simulink model "Quadcopter_v5_1_full"  (R2021a)
settings: Solver=ode4  StartTime=0.0  StopTime=87  FixedStep=0.001  RelTol=1e-6
values from neighbouring files (symbols this model uses):
  mean_wind = [2.72 , 1.75, -0.006]    [main_run.m]    (also in main_run_5_1.m; param_est.m = [2.72 , 1.75, .006])
  q = X(7:10)    [EKF_without_wind.m]
  r = linspace(floor(nr*0.01)/nr,1,nr)    [main_run.m]    (also in main_run_5_1.m)
  w1 = w(1)    [EKF_without_wind.m]
  x0 = [0,0,0,1,0,0,0,-P.mean_wind,0,0,0]    [main_run.m]    (also in main_run_5_1.m)
  xref = [1,1,-8,1,0,0,0,-P.mean_wind]    [main_run.m]    (also in main_run_5_1.m)
undefined symbols (not defined in the file or in its folder): HDBK, MIL, Moderate, P, u1, v1
libraries: simulink x1, aerolibwind2 x1
(part 3 of 6)

== matlab function Quadcopter_v5_1_full/Controller /State Dependent LQR/LQR ==
  data: x input; r input; y output; P parameter; u_c input; t input
function y  = LQR_state(x, r,P,u_c, t)
%State dependent LQR 

  %inputs
  %x---states; this will give all states, f_c and omega
  %prev_state---states from last time step
  %sumError-- not need
  %ref--- reference
y=zeros(4,1);


K0=zeros(4,10);
coder.extrinsic('lqr')

xref= r(1:10);
x_c=x(1:10);
uref = P.uref;


D = P.D;
m = P.m;

p = reshape(x_c(1:3),[3 1]);
q = reshape(x_c(4:7),[4 1]);
v = reshape(x_c(8:10),[3 1]);
nq = norm(q);
% q*q.'
ddqu_dq = (eye(4) - (nq^-2)*q*q.')*(nq^-1) ;

if t==0
    c = uref(4);
    wx = uref(1);
    wy = uref(2);
    wz = uref(3);
else
    c = u_c(4);
    wx = u_c(1);
    wy = u_c(2);
    wz = u_c(3);

end 


qw = q(1);
qx = q(2);
qy = q(3);
qz = q(4);

ddp_dv = eye([3 3]);
ddq_dq = 0.5*[ 0, -wx, -wy, -wz;...
              wx,   0,  wz, -wy;...
              wy, -wz,   0,  wx;...
              wz,  wy, -wx,   0]*ddqu_dq;
ddq_dw = 0.5*[-qx, -qy, -qz;...
               qw, -qz, -qy;...
               qz,  qw,  qx;...
              -qy,  qx,  qw];
ddc_dq = 2*c*[ qy,  qz,  qw, qx;...
              -qx, -qw,  qz, qy;...
               qw, -qx, -qy, qz]*ddqu_dq;
ddv_dc = -[            qw*qy + qx*qz;...
                      qy*qz - qw*qx;...
          qw^2 - qx^2 - qy^2 + qz^2]; 
      
R=quater_rot(q);

% ddrg_v= -(R*D*R'*(norm(v)*eye(3)+(v*v')/norm(v)))/m; %also jacobian of vdot wrt v     
% vx=v(1);
% vy=v(2);
% vz=v(3);
% dx=D(1);
% dy=D(2);
% dz=D(3);
% ddrg_q=[ ((qw^2/(abs(qw)^2 + abs(qx)^2 + abs(qy)^2 + abs(qz)^2) - 1)*(vy*(2*dy*qw*(2*qw*qz - 2*qx*qy)*(abs(vx)^2 + abs(vy)^2 + abs(vz)^2)^(1/2) - 2*dx*qw*(2*qw*qz + 2*qx*qy)*(abs(vx)^2 + abs(vy)^2 + abs(vz)^2)^(1/2) + 2*dz*qx*(2*qw*qy + 2*qx*qz)*(abs(vx)^2 + abs(vy)^2 + abs(vz)^2)^(1/2) + 2*dz*qy*(2*qw*qx - 2*qy*qz)*(abs(vx)^2 + abs(vy)^2 + abs(vz)^2)^(1/2) - 2*dx*qz*(abs(vx)^2 + abs(vy)^2 + abs(vz)^2)^(1/2)*(qw^2 + qx^2 - qy^2 - qz^2) + 2*dy*qz*(abs(vx)^2 + abs(vy)^2 + abs(vz)^2)^(1/2)*(qw^2 - qx^2 + qy^2 - qz^2)) + vz*(2*dx*qw*(2*qw*qy - 2*qx*qz)*(abs(vx)^2 + abs(vy)^2 + abs(vz)^2)^(1/2) + 2*dy*qx*(2*qw*qz - 2*qx*qy)*(abs(vx)^2 + abs(vy)^2 + abs(vz)^2)^(1/2) - 2*dz*qw*(2*qw*qy + 2*qx*qz)*(abs(vx)^2 + abs(vy)^2 + abs(vz)^2)^(1/2) + 2*dy*qz*(2*qw*qx + 2*qy*qz)*(abs(vx)^2 + abs(vy)^2 + abs(vz)^2)^(1/2) + 2*dx*qy*(abs(vx)^2 + abs(vy)^2 + abs(vz)^2)^(1/2)*(qw^2 + qx^2 - qy^2 - qz^2) - 2*dz*qy*(abs(vx)^2 + abs(vy)^2 + abs(vz)^2)^(1/2)*(qw^2 - qx^2 - qy^2 + qz^2)) - vx*(4*dy*qz*(2*qw*qz - 2*qx*qy)*(abs(vx)^2 + abs(vy)^2 + abs(vz)^2)^(1/2) + 4*dz*qy*(2*qw*qy + 2*qx*qz)*(abs(vx)^2 + abs(vy)^2 + abs(vz)^2)^(1/2) + 4*dx*qw*(abs(vx)^2 + abs(vy)^2 + abs(vz)^2)^(1/2)*(qw^2 + qx^2 - qy^2 - qz^2))))/(abs(qw)^2 + abs(qx)^2 + abs(qy)^2 + abs(qz)^2)^(1/2) + (qw*qy*(vy*(2*dx*qy*(2*qw*qz + 2*qx*qy)*(abs(vx)^2 + abs(vy)^2 + abs(vz)^2)^(1/2) + 2*dz*qw*(2*qw*qx - 2*qy*qz)*(abs(vx)^2 + abs(vy)^2 + abs(vz)^2)^(1/2) + 2*dy*qy*(2*qw*qz - 2*qx*qy)*(abs(vx)^2 + abs(vy)^2 + abs(vz)^2)^(1/2) - 2*dz*qz*(2*qw*qy + 2*qx*qz)*(abs(vx)^2 + abs(vy)^2 + abs(vz)^2)^(1/2) - 2*dx*qx*(abs(vx)^2 + abs(vy)^2 + abs(vz)^2)^(1/2)*(qw^2 + qx^2 - qy^2 - qz^2) - 2*dy*qx*(abs(vx)^2 + abs(vy)^2 + abs(vz)^2)^(1/2)*(qw^2 - qx^2 + qy^2 - qz^2)) - vz*(2*dx*qy*(2*qw*qy - 2*qx*qz)*(abs(vx)^2 + abs(vy)^2 + abs(vz)^2)^(1/2) + 2*dy*qx*(2*qw*qx + 2*qy*qz)*(abs(vx)^2 + abs(vy)^2 + abs(vz)^2)^(1/2) - 2*dy*qz*(2*qw*qz - 2*qx*qy)*(abs(vx)^2 + abs(vy)^2 + abs(vz)^2)^(1/2) - 2*dz*qy*(2*qw*qy + 2*qx*qz)*(abs(vx)^2 + abs(vy)^2 + abs(vz)^2)^(1/2) - 2*dx*qw*(abs(vx)^2 + abs(vy)^2 + abs(vz)^2)^(1/2)*(qw^2 + qx^2 - qy^2 - qz^2) + 2*dz*qw*(abs(vx)^2 + abs(vy)^2 + abs(vz)^2)^(1/2)*(qw^2 - qx^2 - qy^2 + qz^2)) + vx*(4*dy*qx*(2*qw*qz - 2*qx*qy)*(abs(vx)^2 + abs(vy)^2 + abs(vz)^2)^(1/2) - 4*dz*qw*(2*qw*qy + 2*qx*qz)*(abs(vx)^2 + abs(vy)^2 + abs(vz)^2)^(1/2) + 4*dx*qy*(abs(vx)^2 + abs(vy)^2 + abs(vz)^2)^(1/2)*(qw^2 + qx^2 - qy^2 - qz^2))))/(abs(qw)^2 + abs(qx)^2 + abs(qy)^2 + abs(qz)^2)^(3/2) - (qw*qx*(vy*(2*dx*qx*(2*qw*qz + 2*qx*qy)*(abs(vx)^2 + abs(vy)^2 + abs(vz)^2)^(1/2) + 2*dy*qx*(2*qw*qz - 2*qx*qy)*(abs(vx)^2 + abs(vy)^2 + abs(vz)^2)^(1/2) - 2*dz*qw*(2*qw*qy + 2*qx*qz)*(abs(vx)^2 + abs(vy)^2 + abs(vz)^2)^(1/2) - 2*dz*qz*(2*qw*qx - 2*qy*qz)*(abs(vx)^2 + abs(vy)^2 + abs(vz)^2)^(1/2) + 2*dx*qy*(abs(vx)^2 + abs(vy)^2 + abs(vz)^2)^(1/2)*(qw^2 + qx^2 - qy^2 - qz^2) + 2*dy*qy*(abs(vx)^2 + abs(vy)^2 + abs(vz)^2)^(1/2)*(qw^2 - qx^2 + qy^2 - qz^2)) - vz*(2*dx*qx*(2*qw*qy - 2*qx*qz)*(abs(vx)^2 + abs(vy)^2 + abs(vz)^2)^(1/2) + 2*dy*qw*(2*qw*qz - 2*qx*qy)*(abs(vx)^2 + abs(vy)^2 + abs(vz)^2)^(1/2) - 2*dy*qy*(2*qw*qx + 2*qy*qz)*(abs(vx)^2 + abs(vy)^2 + abs(vz)^2)^(1/2) + 2*dz*qx*(2*qw*qy + 2*qx*qz)*(abs(vx)^2 + abs(vy)^2 + abs(vz)^2)^(1/2) - 2*dx*qz*(abs(vx)^2 + abs(vy)^2 + abs(vz)^2)^(1/2)*(qw^2 + qx^2 - qy^2 - qz^2) - 2*dz*qz*(abs(vx)^2 + abs(vy)^2 + abs(vz)^2)^(1/2)*(qw^2 - qx^2 - qy^2 + qz^2)) + vx*(4*dz*qz*(2*qw*qy + 2*qx*qz)*(abs(vx)^2 + abs(vy)^2 + abs(vz)^2)^(1/2) - 4*dy*qy*(2*qw*qz - 2*qx*qy)*(abs(vx)^2 + abs(vy)^2 + abs(vz)^2)^(1/2) + 4*dx*qx*(abs(vx)^2 + abs(vy)^2 + abs(vz)^2)^(1/2)*(qw^2 + qx^2 - qy^2 - qz^2))))/(abs(qw)^2 + abs(qx)^2 + abs(qy)^2 + abs(qz)^2)^(3/2) - (qw*qz*(vz*(2*dx*qz*(2*qw*qy - 2*qx*qz)*(abs(vx)^2 + abs(vy)^2 + abs(vz)^2)^(1/2) - 2*dy*qw*(2*qw*qx + 2*qy*qz)*(abs(vx)^2 + abs(vy)^2 + abs(vz)^2)^(1/2) - 2*dy*qy*(2*qw*qz - 2*qx*qy)*(abs(vx)^2 + abs(vy)^2 + abs(vz)^2)^(1/2) + 2*dz*qz*(2*qw*qy + 2*qx*qz)*(abs(vx)^2 + abs(vy)^2 + abs(vz)^2)^(1/2) + 2*dx*qx*(abs(vx)^2 + abs(vy)^2 + abs(vz)^2)^(1/2)*(qw^2 + qx^2 - qy^2 - qz^2) + 2*dz*qx*(abs(vx)^2 + abs(vy)^2 + abs(vz)^2)^(1/2)*(qw^2 - qx^2 - qy^2 + qz^2)) - vy*(2*dx*qz*(2*qw*qz + 2*qx*qy)*(abs(vx)^2 + abs(vy)^2 + abs(vz)^2)^(1/2) + 2*dz*qx*(2*qw*qx - 2*qy*qz)*(abs(vx)^2 + abs(vy)^2 + abs(vz)^2)^(1/2) - 2*dy*qz*(2*qw*qz - 2*qx*qy)*(abs(vx)^2 + abs(vy)^2 + abs(vz)^2)^(1/2) - 2*dz*qy*(2*qw*qy + 2*qx*qz)*(abs(vx)^2 + abs(vy)^2 + abs(vz)^2)^(1/2) - 2*dx*qw*(abs(vx)^2 + abs(vy)^2 + abs(vz)^2)^(1/2)*(qw^2 + qx^2 - qy^2 - qz^2) + 2*dy*qw*(abs(vx)^2 + abs(vy)^2 + abs(vz)^2)^(1/2)*(qw^2 - qx^2 + qy^2 - qz^2)) + vx*(4*dy*qw*(2*qw*qz - 2*qx*qy)*(abs(vx)^2 + abs(vy)^2 + abs(vz)^2)^(1/2) + 4*dz*qx*(2*qw*qy + 2*qx*qz)*(abs(vx)^2 + abs(vy)^2 + abs(vz)^2)^(1/2) - 4*dx*qz*(abs(vx)^2 + abs(vy)^2 + abs(vz)^2)^(1/2)*(qw^2 + qx^2 - qy^2 - qz^2))))/(abs(qw)^2 + abs(qx)^2 + abs(qy)^2 + abs(qz)^2)^(3/2), (qw*qx*(vy*(2*dy*qw*(2*qw*qz - 2*qx*qy)*(abs(vx)^2 + abs(vy)^2 + abs(vz)^2)^(1/2) - 2*dx*qw*(2*qw*qz + 2*qx*qy)*(abs(vx)^2 + abs(vy)^2 + abs(vz)^2)^(1/2) + 2*dz*qx*(2*qw*qy + 2*qx*qz)*(abs(vx)^2 + abs(vy)^2 + abs(vz)^2)^(1/2) + 2*dz*qy*(2*qw*qx - 2*qy*qz)*(abs(vx)^2 + abs(vy)^2 + abs(vz)^2)^(1/2) - 2*dx*qz*(abs(vx)^2 + abs(vy)^2 + abs(vz)^2)^(1/2)*(qw^2 + qx^2 - qy^2 - qz^2) + 2*dy*qz*(abs(vx)^2 + abs(vy)^2 + abs(vz)^2)^(1/2)*(qw^2 - qx^2 + qy^2 - qz^2)) + vz*(2*dx*qw*(2*qw*qy - 2*qx*qz)*(abs(vx)^2 + abs(vy)^2 + abs(vz)^2)^(1/2) + 2*dy*qx*(2*qw*qz - 2*qx*qy)*(abs(vx)^2 + abs(vy)^2 + abs(vz)^2)^(1/2) - 2*dz*qw*(2*qw*qy + 2*qx*qz)*(abs(vx)^2 + abs(vy)^2 + abs(vz)^2)^(1/2) + 2*dy*qz*(2*qw*qx + 2*qy*qz)*(abs(vx)^2 + abs(vy)^2 + abs(vz)^2)^(1/2) + 2*dx*qy*(abs(vx)^2 + abs(vy)^2 + abs(vz)^2)^(1/2)*(qw^2 + qx^2 - qy^2 - qz^2) - 2*dz*qy*(abs(vx)^2 + abs(vy)^2 + abs(vz)^2)^(1/2)*(qw^2 - qx^2 - qy^2 + qz^2)) - vx*(4*dy*qz*(2*qw*qz - 2*qx*qy)*(abs(vx)^2 + abs(vy)^2 + abs(vz)^2)^(1/2) + 4*dz*qy*(2*qw*qy + 2*qx*qz)*(abs(vx)^2 + abs(vy)^2 + abs(vz)^2)^(1/2) + 4*dx*qw*(abs(vx)^2 + abs(vy)^2 + abs(vz)^2)^(1/2)*(qw^2 + qx^2 - qy^2 - qz^2))))/(abs(qw)^2 + abs(qx)^2 + abs(qy)^2 + abs(qz)^2)^(3/2) - ((qx^2/(abs(qw)^2 + abs(qx)^2 + abs(qy)^2 + abs(qz)^2) - 1)*(vy*(2*dx*qx*(2*qw*qz + 2*qx*qy)*(abs(vx)^2 + abs(vy)^2 + abs(vz)^2)^(1/2) + 2*dy*qx*(2*qw*qz - 2*qx*qy)*(abs(vx)^2 + abs(vy)^2 + abs(vz)^2)^(1/2) - 2*dz*qw*(2*qw*qy + 2*qx*qz)*(abs(vx)^2 + abs(vy)^2 + abs(vz)^2)^(1/2) - 2*dz*qz*(2*qw*qx - 2*qy*qz)*(abs(vx)^2 + abs(vy)^2 + abs(vz)^2)^(1/2) + 2*dx*qy*(abs(vx)^2 + abs(vy)^2 + abs(vz)^2)^(1/2)*(qw^2 + qx^2 - qy^2 - qz^2) + 2*dy*qy*(abs(vx)^2 + abs(vy)^2 + abs(vz)^2)^(1/2)*(qw^2 - qx^2 + qy^2 - qz^2)) - vz*(2*dx*qx*(2*qw*qy - 2*qx*qz)*(abs(vx)^2 + abs(vy)^2 + abs(vz)^2)^(1/2) + 2*dy*qw*(2*qw*qz - 2*qx*qy)*(abs(vx)^2 + abs(vy)^2 + abs(vz)^2)^(1/2) - 2*dy*qy*(2*qw*qx + 2*qy*qz)*(abs(vx)^2 + abs(vy)^2 + abs(vz)^2)^(1/2) + 2*dz*qx*(2*qw*qy + 2*qx*qz)*(abs(vx)^2 + abs(vy)^2 + abs(vz)^2)^(1/2) - 2*dx*qz*(abs(vx)^2 + abs(vy)^2 + abs(vz)^2)^(1/2)*(qw^2 + qx^2 - qy^2 - qz^2) - 2*dz*qz*(abs(vx)^2 + abs(vy)^2 + abs(vz)^2)^(1/2)*(qw^2 - qx^2 - qy^2 + qz^2)) + vx*(4*dz*qz*(2*qw*qy + 2*qx*qz)*(abs(vx)^2 + abs(vy)^2 + abs(vz)^2)^(1/2) - 4*dy*qy*(2*qw*qz - 2*qx*qy)*(abs(vx)^2 + abs(vy)^2 + abs(vz)^2)^(1/2) + 4*dx*qx*(abs(vx)^2 + abs(vy)^2 + abs(vz)^2)^(1/2)*(qw^2 + qx^2 - qy^2 - qz^2))))/(abs(qw)^2 + abs(qx)^2 + abs(qy)^2 + abs(qz)^2)^(1/2) + (qx*qy*(vy*(2*dx*qy*(2*qw*qz + 2*qx*qy)*(abs(vx)^2 + abs(vy)^2 + abs(vz)^2)^(1/2) + 2*dz*qw*(2*qw*qx - 2*qy*qz)*(abs(vx)^2 + abs(vy)^2 + abs(vz)^2)^(1/2) + 2*dy*qy*(2*qw*qz - 2*qx*qy)*(abs(vx)^2 + abs(vy)^2 + abs(vz)^2)^(1/2) - 2*dz*qz*(2*qw*qy + 2*qx*qz)*(abs(vx)^2 + abs(vy)^2 + abs(vz)^2)^(1/2) - 2*dx*qx*(abs(vx)^2 + abs(vy)^2 + abs(vz)^2)^(1/2)*(qw^2 + qx^2 - qy^2 - qz^2) - 2*dy*qx*(abs(vx)^2 + abs(vy)^2 + abs(vz)^2)^(1/2)*(qw^2 - qx^2 + qy^2 - qz^2)) - vz*(2*dx*qy*(2*qw*qy - 2*qx*qz)*(abs(vx)^2 + abs(vy)^2 + abs(vz)^2)^(1/2) + 2*dy*qx*(2*qw*qx + 2*qy*qz)*(abs(vx)^2 + abs(vy)^2 + abs(vz)^2)^(1/2) - 2*dy*qz*(2*qw*qz - 2*qx*qy)*(abs(vx)^2 + abs(vy)^2 + abs(vz)^2)^(1/2) - 2*dz*qy*(2*qw*qy + 2*qx*qz)*(abs(vx)^2 + abs(vy)^2 + abs(vz)^2)^(1/2) - 2*dx*qw*(abs(vx)^2 + abs(vy)^2 + abs(vz)^2)^(1/2)*(qw^2 + qx^2 - qy^2 - qz^2) + 2*dz*qw*(abs(vx)^2 + abs(vy)^2 + abs(vz)^2)^(1/2)*(qw^2 - qx^2 - qy^2 + qz^2)) + vx*(4*dy*qx*(2*qw*qz - 2*qx*qy)*(abs(vx)^2 + abs(vy)^2 + abs(vz)^2)^(1/2) - 4*dz*qw*(2*qw*qy + 2*qx*qz)*(abs(vx)^2 + abs(vy)^2 + abs(vz)^2)^(1/2) + 4*dx*qy*(abs(vx)^2 + abs(vy)^2 + abs(vz)^2)^(1/2)*(qw^2 + qx^2 - qy^2 - qz^2))))/(abs(qw)^2 + abs(qx)^2 + abs(qy)^2 + abs(qz)^2)^(3/2) - (qx*qz*(vz*(2*dx*qz*(2*qw*qy - 2*qx*qz)*(abs(vx)^2 + abs(vy)^2 + abs(vz)^2)^(1/2) - 2*dy*qw*(2*qw*qx + 2*qy*qz)*(abs(vx)^2 + abs(vy)^2 + abs(vz)^2)^(1/2) - 2*dy*qy*(2*qw*qz - 2*qx*qy)*(abs(vx)^2 + abs(vy)^2 + abs(vz)^2)^(1/2) + 2*dz*qz*(2*qw*qy + 2*qx*qz)*(abs(vx)^2 + abs(vy)^2 + abs(vz)^2)^(1/2) + 2*dx*qx*(abs(vx)^2 + abs(vy)^2 + abs(vz)^2)^(1/2)*(qw^2 + qx^2 - qy^2 - qz^2) + 2*dz*qx*(abs(vx)^2 + abs(vy)^2 + abs(vz)^2)^(1/2)*(qw^2 - qx^2 - qy^2 + qz^2)) - vy*(2*dx*qz*(2*qw*qz + 2*qx*qy)*(abs(vx)^2 + abs(vy)^2 + abs(vz)^2)^(1/2) + 2*dz*qx*(2*qw*qx - 2*qy*qz)*(abs(vx)^2 + abs(vy)^2 + abs(vz)^2)^(1/2) - 2*dy*qz*(2*qw*qz - 2*qx*qy)*(abs(vx)^2 + abs(vy)^2 + abs(vz)^2)^(1/2) - 2*dz*qy*(2*qw*qy + 2*qx*qz)*(abs(vx)^2 + abs(vy)^2 + abs(vz)^2)^(1/2) - 2*dx*qw*(abs(vx)^2 + abs(vy)^2 + abs(vz)^2)^(1/2)*(qw^2 + qx^2 - qy^2 - qz^2) + 2*dy*qw*(abs(vx)^2 + abs(vy)^2 + abs(vz)^2)^(1/2)*(qw^2 - qx^2 + qy^2 - qz^2)) + vx*(4*dy*qw*(2*qw*qz - 2*qx*qy)*(abs(vx)^2 + abs(vy)^2 + abs(vz)^2)^(1/2) + 4*dz*qx*(2*qw*qy + 2*qx*qz)*(abs(vx)^2 + abs(vy)^2 + abs(vz)^2)^(1/2) - 4*dx*qz*(abs(vx)^2 + abs(vy)^2 + abs(vz)^2)^(1/2)*(qw^2 + qx^2 - qy^2 - qz^2))))/(abs(qw)^2 + abs(qx)^2 + abs(qy)^2 + abs(qz)^2)^(3/2), ((qy^2/(abs(qw)^2 + abs(qx)^2 + abs(qy)^2 + abs(qz)^2) - 1)*(vy*(2*dx*qy*(2*qw*qz + 2*qx*qy)*(abs(vx)^2 + abs(vy)^2 + abs(vz)^2)^(1/2) + 2*dz*qw*(2*qw*qx - 2*qy*qz)*(abs(vx)^2 + abs(vy)^2 + abs(vz)^2)^(1/2) + 2*dy*qy*(2*qw*qz - 2*qx*qy)*(abs(vx)^2 + abs(vy)^2 + abs(vz)^2)^(1/2) - 2*dz*qz*(2*qw*qy + 2*qx*qz)*(abs(vx)^2 + abs(vy)^2 + abs(vz)^2)^(1/2) - 2*dx*qx*(abs(vx)^2 + abs(vy)^2 + abs(vz)^2)^(1/2)*(qw^2 + qx^2 - qy^2 - qz^2) - 2*dy*qx*(abs(vx)^2 + abs(vy)^2 + abs(vz)^2)^(1/2)*(qw^2 - qx^2 + qy^2 - qz^2)) - vz*(2*dx*qy*(2*qw*qy - 2*qx*qz)*(abs(vx)^2 + abs(vy)^2 + abs(vz)^2)^(1/2) + 2*dy*qx*(2*qw*qx + 2*qy*qz)*(abs(vx)^2 + abs(vy)^2 + abs(vz)^2)^(1/2) - 2*dy*qz*(2*qw*qz - 2*qx*qy)*(abs(vx)^2 + abs(vy)^2 + abs(vz)^2)^(1/2) - 2*dz*qy*(2*qw*qy + 2*qx*qz)*(abs(vx)^2 + abs(vy)^2 + abs(vz)^2)^(1/2) - 2*dx*qw*(abs(vx)^2 + abs(vy)^2 + abs(vz)^2)^(1/2)*(qw^2 + qx^2 - qy^2 - qz^2) + 2*dz*qw*(abs(vx)^2 + abs(vy)^2 + abs(vz)^2)^(1/2)*(qw^2 - qx^2 - qy^2 + qz^2)) + vx*(4*dy*qx*(2*qw*qz - 2*qx*qy)*(abs(vx)^2 + abs(vy)^2 + abs(vz)^2)^(1/2) - 4*dz*qw*(2*qw*qy + 2*qx*qz)*(abs(vx)^2 + abs(vy)^2 + abs(vz)^2)^(1/2) + 4*dx*qy*(abs(vx)^2 + abs(vy)^2 + abs(vz)^2)^(1/2)*(qw^2 + qx^2 - qy^2 - qz^2))))/(abs(qw)^2 + abs(qx)^2 + abs(qy)^2 + abs(qz)^2)^(1/2) + (qw*qy*(vy*(2*dy*qw*(2*qw*qz - 2*qx*qy)*(abs(vx)^2 + abs(vy)^2 + abs(vz)^2)^(1/2) - 2*dx*qw*(2*qw*qz + 2*qx*qy)*(abs(vx)^2 + abs(vy)^2 + abs(vz)^2)^(1/2) + 2*dz*qx*(2*qw*qy + 2*qx*qz)*(abs(vx)^2 + abs(vy)^2 + abs(vz)^2)^(1/2) + 2*dz*qy*(2*qw*qx - 2*qy*qz)*(abs(vx)^2 + abs(vy)^2 + abs(vz)^2)^(1/2) - 2*dx*qz*(abs(vx)^2 + abs(vy)^2 + abs(vz)^2)^(1/2)*(qw^2 + qx^2 - qy^2 - qz^2) + 2*dy*qz*(abs(vx)^2 + abs(vy)^2 + abs(vz)^2)^(1/2)*(qw^2 - qx^2 + qy^2 - qz^2)) + vz*(2*dx*qw*(2*qw*qy - 2*qx*qz)*(abs(vx)^2 + abs(vy)^2 + abs(vz)^2)^(1/2) + 2*dy*qx*(2*qw*qz - 2*qx*qy)*(abs(vx)^2 + abs(vy)^2 + abs(vz)^2)^(1/2) - 2*dz*qw*(2*qw*qy + 2*qx*qz)*(abs(vx)^2 + abs(vy)^2 + abs(vz)^2)^(1/2) + 2*dy*qz*(2*qw*qx + 2*qy*qz)*(abs(vx)^2 + abs(vy)^2 + abs(vz)^2)^(1/2) + 2*dx*qy*(abs(vx)^2 + abs(vy)^2 + abs(vz)^2)^(1/2)*(qw^2 + qx^2 - qy^2 - qz^2) - 2*dz*qy*(abs(vx)^2 + abs(vy)^2 + abs(vz)^2)^(1/2)*(qw^2 - qx^2 - qy^2 + qz^2)) - vx*(4*dy*qz*(2*qw*qz - 2*qx*qy)*(abs(vx)^2 + abs(vy)^2 + abs(vz)^2)^(1/2) + 4*dz*qy*(2*qw*qy + 2*qx*qz)*(abs(vx)^2 + abs(vy)^2 + abs(vz)^2)^(1/2) + 4*dx*qw*(abs(vx)^2 + abs(vy)^2 + abs(vz)^2)^(1/2)*(qw^2 + qx^2 - qy^2 - qz^2))))/(abs(qw)^2 + abs(qx)^2 + abs(qy)^2 + abs(qz)^2)^(3/2) - (qx*qy*(vy*(2*dx*qx*(2*qw*qz + 2*qx*qy)*(abs(vx)^2 + abs(vy)^2 + abs(vz)^2)^(1/2) + 2*dy*qx*(2*qw*qz - 2*qx*qy)*(abs(vx)^2 + abs(vy)^2 + abs(vz)^2)^(1/2) - 2*dz*qw*(2*qw*qy + 2*qx*qz)*(abs(vx)^2 + abs(vy)^2 + abs(vz)^2)^(1/2) - 2*dz*qz*(2*qw*qx - 2*qy*qz)*(abs(vx)^2 + abs(vy)^2 + abs(vz)^2)^(1/2) + 2*dx*qy*(abs(vx)^2 + abs(vy)^2 + abs(vz)^2)^(1/2)*(qw^2 + qx^2 - qy^2 - qz^2) + 2*dy*qy*(abs(vx)^2 + abs(vy)^2 + abs(vz)^2)^(1/2)*(qw^2 - qx^2 + qy^2 - qz^2)) - vz*(2*dx*qx*(2*qw*qy - 2*qx*qz)*(abs(vx)^2 + abs(vy)^2 + abs(vz)^2)^(1/2) + 2*dy*qw*(2*qw*qz - 2*qx*qy)*(abs(vx)^2 + abs(vy)^2 + abs(vz)^2)^(1/2) - 2*dy*qy*(2*qw*qx + 2*qy*qz)*(abs(vx)^2 + abs(vy)^2 + abs(vz)^2)^(1/2) + 2*dz*qx*(2*qw*qy + 2*qx*qz)*(abs(vx)^2 + abs(vy)^2 + abs(vz)^2)^(1/2) - 2*dx*qz*(abs(vx)^2 + abs(vy)^2 + abs(vz)^2)^(1/2)*(qw^2 + qx^2 - qy^2 - qz^2) - 2*dz*qz*(abs(vx)^2 + abs(vy)^2 + abs(vz)^2)^(1/2)*(qw^2 - qx^2 - qy^2 + qz^2)) + vx*(4*dz*qz*(2*qw*qy + 2*qx*qz)*(abs(vx)^2 + abs(vy)^2 + abs(vz)^2)^(1/2) - 4*dy*qy*(2*qw*qz - 2*qx*qy)*(abs(vx)^2 + abs(vy)^2 + abs(vz)^2)^(1/2) + 4*dx*qx*(abs(vx)^2 + abs(vy)^2 + abs(vz)^2)^(1/2)*(qw^2 + qx^2 - qy^2 - qz^2))))/(abs(qw)^2 + abs(qx)^2 + abs(qy)^2 + abs(qz)^2)^(3/2) - (qy*qz*(vz*(2*dx*qz*(2*qw*qy - 2*qx*qz)*(abs(vx)^2 + abs(vy)^2 + abs(vz)^2)^(1/2) - 2*dy*qw*(2*qw*qx + 2*qy*qz)*(abs(vx)^2 + abs(vy)^2 + abs(vz)^2)^(1/2) - 2*dy*qy*(2*qw*qz - 2*qx*qy)*(abs(vx)^2 + abs(vy)^2 + abs(vz)^2)^(1/2) + 2*dz*qz*(2*qw*qy + 2*qx*qz)*(abs(vx)^2 + abs(vy)^2 + abs(vz)^2)^(1/2) + 2*dx*qx*(abs(vx)^2 + abs(vy)^2 + abs(vz)^2)^(1/2)*(qw^2 + qx^2 - qy^2 - qz^2) + 2*dz*qx*(abs(vx)^2 + abs(vy)^2 + abs(vz)^2)^(1/2)*(qw^2 - qx^2 - qy^2 + qz^2)) - vy*(2*dx*qz*(2*qw*qz + 2*qx*qy)*(abs(vx)^2 + abs(vy)^2 + abs(vz)^2)^(1/2) + 2*dz*qx*(2*qw*qx - 2*qy*qz)*(abs(vx)^2 + abs(vy)^2 + abs(vz)^2)^(1/2) - 2*dy*qz*(2*qw*qz - 2*qx*qy)*(abs(vx)^2 + abs(vy)^2 + abs(vz)^2)^(1/2) - 2*dz*qy*(2*qw*qy + 2*qx*qz)*(abs(vx)^2 + abs(vy)^2 + abs(vz)^2)^(1/2) - 2*dx*qw*(abs(vx)^2 + abs(vy)^2 + abs(vz)^2)^(1/2)*(qw^2 + qx^2 - qy^2 - qz^2) + 2*dy*qw*(abs(vx)^2 + abs(vy)^2 + abs(vz)^2)^(1/2)*(qw^2 - qx^2 + qy^2 - qz^2)) + vx*(4*dy*qw*(2*qw*qz - 2*qx*qy)*(abs(vx)^2 + abs(vy)^2 + abs(vz)^2)^(1/2) + 4*dz*qx*(2*qw*qy + 2*qx*qz)*(abs(vx)^2 + abs(vy)^2 + abs(vz)^2)^(1/2) - 4*dx*qz*(abs(vx)^2 + abs(vy)^2 + abs(vz)^2)^(1/2)*(qw^2 + qx^2 - qy^2 - qz^2))))/(abs(qw)^2 + abs(qx)^2 + abs(qy)^2 + abs(qz)^2)^(3/2), (qw*qz*(vy*(2*dy*qw*(2*qw*qz - 2*qx*qy)*(abs(vx)^2 + abs(vy)^2 + abs(vz)^2)^(1/2) - 2*dx*qw*(2*qw*qz + 2*qx*qy)*(abs(vx)^2 + abs(vy)^2 + abs(vz)^2)^(1/2) + 2*dz*qx*(2*qw*qy + 2*qx*qz)*(abs(vx)^2 + abs(vy)^2 + abs(vz)^2)^(1/2) + 2*dz*qy*(2*qw*qx - 2*qy*qz)*(abs(vx)^2 + abs(vy)^2 + abs(vz)^2)^(1/2) - 2*dx*qz*(abs(vx)^2 + abs(vy)^2 + abs(vz)^2)^(1/2)*(qw^2 + qx^2 - qy^2 - qz^2) + 2*dy*qz*(abs(vx)^2 + abs(vy)^2 + abs(vz)^2)^(1/2)*(qw^2 - qx^2 + qy^2 - qz^2)) + vz*(2*dx*qw*(2*qw*qy - 2*qx*qz)*(abs(vx)^2 + abs(vy)^2 + abs(vz)^2)^(1/2) + 2*dy*qx*(2*qw*qz - 2*qx*qy)*(abs(vx)^2 + abs(vy)^2 + abs(vz)^2)^(1/2) - 2*dz*qw*(2*qw*qy + 2*qx*qz)*(abs(vx)^2 + abs(vy)^2 + abs(vz)^2)^(1/2) + 2*dy*qz*(2*qw*qx + 2*qy*qz)*(abs(vx)^2 + abs(vy)^2 + abs(vz)^2)^(1/2) + 2*dx*qy*(abs(vx)^2 + abs(vy)^2 + abs(vz)^2)^(1/2)*(qw^2 + qx^2 - qy^2 - qz^2) - 2*dz*qy*(abs(vx)^2 + abs(vy)^2 + abs(vz)^2)^(1/2)*(qw^2 - qx^2 - qy^2 + qz^2)) - vx*(4*dy*qz*(2*qw*qz - 2*qx*qy)*(abs(vx)^2 + abs(vy)^2 + abs(vz)^2)^(1/2) + 4*dz*qy*(2*qw*qy + 2*qx*qz)*(abs(vx)^2 + abs(vy)^2 + abs(vz)^2)^(1/2) + 4*dx*qw*(abs(vx)^2 + abs(vy)^2 + abs(vz)^2)^(1/2)*(qw^2 + qx^2 - qy^2 - qz^2))))/(abs(qw)^2 + abs(qx)^2 + abs(qy)^2 + abs(qz)^2)^(3/2) - ((qz^2/(abs(qw)^2 + abs(qx)^2 + abs(qy)^2 + abs(qz)^2) - 1)*(vz*(2*dx*qz*(2*qw*qy - 2*qx*qz)*(abs(vx)^2 + abs(vy)^2 + abs(vz)^2)^(1/2) - 2*dy*qw*(2*qw*qx + 2*qy*qz)*(abs(vx)^2 + abs(vy)^2 + abs(vz)^2)^(1/2) - 2*dy*qy*(2*qw*qz - 2*qx*qy)*(abs(vx)^2 + abs(vy)^2 + abs(vz)^2)^(1/2) + 2*dz*qz*(2*qw*qy + 2*qx*qz)*(abs(vx)^2 + abs(vy)^2 + abs(vz)^2)^(1/2) + 2*dx*qx*(abs(vx)^2 + abs(vy)^2 + abs(vz)^2)^(1/2)*(qw^2 + qx^2 - qy^2 - qz^2) + 2*dz*qx*(abs(vx)^2 + abs(vy)^2 + abs(vz)^2)^(1/2)*(qw^2 - qx^2 - qy^2 + qz^2)) - vy*(2*dx*qz*(2*qw*qz + 2*qx*qy)*(abs(vx)^2 + abs(vy)^2 + abs(vz)^2)^(1/2) + 2*dz*qx*(2*qw*qx - 2*qy*qz)*(abs(vx)^2 + abs(vy)^2 + abs(vz)^2)^(1/2) - 2*dy*qz*(2*qw*qz - 2*qx*qy)*(abs(vx)^2 + abs(vy)^2 + abs(vz)^2)^(1/2) - 2*dz*qy*(2*qw*qy + 2*qx*qz)*(abs(vx)^2 + abs(vy)^2 + abs(vz)^2)^(1/2) - 2*dx*qw*(abs(vx)^2 + abs(vy)^2 + abs(vz)^2)^(1/2)*(qw^2 + qx^2 - qy^2 - qz^2) + 2*dy*qw*(abs(vx)^2 + abs(vy)^2 + abs(vz)^2)^(1/2)*(qw^2 - qx^2 + qy^2 - qz^2)) + vx*(4*dy*qw*(2*qw*qz - 2*qx*qy)*(abs(vx)^2 + abs(vy)^2 + abs(vz)^2)^(1/2) + 4*dz*qx*(2*qw*qy + 2*qx*qz)*(abs(vx)^2 + abs(vy)^2 + abs(vz)^2)^(1/2) - 4*dx*qz*(abs(vx)^2 + abs(vy)^2 + abs(vz)^2)^(1/2)*(qw^2 + qx^2 - qy^2 - qz^2))))/(abs(qw)^2 + abs(qx)^2 + abs(qy)^2 + abs(qz)^2)^(1/2) + (qy*qz*(vy*(2*dx*qy*(2*qw*qz + 2*qx*qy)*(abs(vx)^2 + abs(vy)^2 + abs(vz)^2)^(1/2) + 2*dz*qw*(2*qw*qx - 2*qy*qz)*(abs(vx)^2 + abs(vy)^2 + abs(vz)^2)^(1/2) + 2*dy*qy*(2*qw*qz - 2*qx*qy)*(abs(vx)^2 + abs(vy)^2 + abs(vz)^2)^(1/2) - 2*dz*qz*(2*qw*qy + 2*qx*qz)*(abs(vx)^2 + abs(vy)^2 + abs(vz)^2)^(1/2) - 2*dx*qx*(abs(vx)^2 + abs(vy)^2 + abs(vz)^2)^(1/2)*(qw^2 + qx^2 - qy^2 - qz^2) - 2*dy*qx*(abs(vx)^2 + abs(vy)^2 + abs(vz)^2)^(1/2)*(qw^2 - qx^2 + qy^2 - qz^2)) - vz*(2*dx*qy*(2*qw*qy - 2*qx*qz)*(abs(vx)^2 + abs(vy)^2 + abs(vz)^2)^(1/2) + 2*dy*qx*(2*qw*qx + 2*qy*qz)*(abs(vx)^2 + abs(vy)^2 + abs(vz)^2)^(1/2) - 2*dy*qz*(2*qw*qz - 2*qx*qy)*(abs(vx)^2 + abs(vy)^2 + abs(vz)^2)^(1/2) - 2*dz*qy*(2*qw*qy + 2*qx*qz)*(abs(vx)^2 + abs(vy)^2 + abs(vz)^2)^(1/2) - 2*dx*qw*(abs(vx)^2 + abs(vy)^2 + abs(vz)^2)^(1/2)*(qw^2 + qx^2 - qy^2 - qz^2) + 2*dz*qw*(abs(vx)^2 + abs(vy)^2 + abs(vz)^2)^(1/2)*(qw^2 - qx^2 - qy^2 + qz^2)) + vx*(4*dy*qx*(2*qw*qz - 2*qx*qy)*(abs(vx)^2 + abs(vy)^2 + abs(vz)^2)^(1/2) - 4*dz*qw*(2*qw*qy + 2*qx*qz)*(abs(vx)^2 + abs(vy)^2 + abs(vz)^2)^(1/2) + 4*dx*qy*(abs(vx)^2 + abs(vy)^2 + abs(vz)^2)^(1/2)*(qw^2 + qx^2 - qy^2 - qz^2))))/(abs(qw)^2 + abs(qx)^2 + abs(qy)^2 + abs(qz)^2)^(3/2) - (qx*qz*(vy*(2*dx*qx*(2*qw*qz + 2*qx*qy)*(abs(vx)^2 + abs(vy)^2 + abs(vz)^2)^(1/2) + 2*dy*qx*(2*qw*qz - 2*qx*qy)*(abs(vx)^2 + abs(vy)^2 + abs(vz)^2)^(1/2) - 2*dz*qw*(2*qw*qy + 2*qx*qz)*(abs(vx)^2 + abs(vy)^2 + abs(vz)^2)^(1/2) - 2*dz*qz*(2*qw*qx - 2*qy*qz)*(abs(vx)^2 + abs(vy)^2 + abs(vz)^2)^(1/2) + 2*dx*qy*(abs(vx)^2 + abs(vy)^2 + abs(vz)^2)^(1/2)*(qw^2 + qx^2 - qy^2 - qz^2) + 2*dy*qy*(abs(vx)^2 + abs(vy)^2 + abs(vz)^2)^(1/2)*(qw^2 - qx^2 + qy^2 - qz^2)) - vz*(2*dx*qx*(2*qw*qy - 2*qx*qz)*(abs(vx)^2 + abs(vy)^2 + abs(vz)^2)^(1/2) + 2*dy*qw*(2*qw*qz - 2*qx*qy)*(abs(vx)^2 + abs(vy)^2 + abs(vz)^2)^(1/2) - 2*dy*qy*(2*qw*qx + 2*qy*qz)*(abs(vx)^2 + abs(vy)^2 + abs(vz)^2)^(1/2) + 2*dz*qx*(2*qw*qy + 2*qx*qz)*(abs(vx)^2 + abs(vy)^2 + abs(vz)^2)^(1/2) - 2*dx*qz*(abs(vx)^2 + abs(vy)^2 + abs(vz)^2)^(1/2)*(qw^2 + qx^2 - qy^2 - qz^2) - 2*dz*qz*(abs(vx)^2 + abs(vy)^2 + abs(vz)^2)^(1/2)*(qw^2 - qx^2 - qy^2 + qz^2)) + vx*(4*dz*qz*(2*qw*qy + 2*qx*qz)*(abs(vx)^2 + abs(vy)^2 + abs(vz)^2)^(1/2) - 4*dy*qy*(2*qw*qz - 2*qx*qy)*(abs(vx)^2 + abs(vy)^2 + abs(vz)^2)^(1/2) + 4*dx*qx*(abs(vx)^2 + abs(vy)^2 + abs(vz)^2)^(1/2)*(qw^2 + qx^2 - qy^2 - qz^2))))/(abs(qw)^2 + abs(qx)^2 + abs(qy)^2 + abs(qz)^2)^(3/2);
% ((qw^2/(abs(qw)^2 + abs(qx)^2 + abs(qy)^2 + abs(qz)^2) - 1)*(vx*(2*dy*qw*(2*qw*qz - 2*qx*qy)*(abs(vx)^2 + abs(vy)^2 + abs(vz)^2)^(1/2) - 2*dx*qw*(2*qw*qz + 2*qx*qy)*(abs(vx)^2 + abs(vy)^2 + abs(vz)^2)^(1/2) + 2*dz*qx*(2*qw*qy + 2*qx*qz)*(abs(vx)^2 + abs(vy)^2 + abs(vz)^2)^(1/2) + 2*dz*qy*(2*qw*qx - 2*qy*qz)*(abs(vx)^2 + abs(vy)^2 + abs(vz)^2)^(1/2) - 2*dx*qz*(abs(vx)^2 + abs(vy)^2 + abs(vz)^2)^(1/2)*(qw^2 + qx^2 - qy^2 - qz^2) + 2*dy*qz*(abs(vx)^2 + abs(vy)^2 + abs(vz)^2)^(1/2)*(qw^2 - qx^2 + qy^2 - qz^2)) + vz*(2*dx*qy*(2*qw*qz + 2*qx*qy)*(abs(vx)^2 + abs(vy)^2 + abs(vz)^2)^(1/2) - 2*dy*qw*(2*qw*qx + 2*qy*qz)*(abs(vx)^2 + abs(vy)^2 + abs(vz)^2)^(1/2) + 2*dz*qw*(2*qw*qx - 2*qy*qz)*(abs(vx)^2 + abs(vy)^2 + abs(vz)^2)^(1/2) + 2*dx*qz*(2*qw*qy - 2*qx*qz)*(abs(vx)^2 + abs(vy)^2 + abs(vz)^2)^(1/2) - 2*dy*qx*(abs(vx)^2 + abs(vy)^2 + abs(vz)^2)^(1/2)*(qw^2 - qx^2 + qy^2 - qz^2) + 2*dz*qx*(abs(vx)^2 + abs(vy)^2 + abs(vz)^2)^(1/2)*(qw^2 - qx^2 - qy^2 + qz^2)) - vy*(4*dx*qz*(2*qw*qz + 2*qx*qy)*(abs(vx)^2 + abs(vy)^2 + abs(vz)^2)^(1/2) + 4*dz*qx*(2*qw*qx - 2*qy*qz)*(abs(vx)^2 + abs(vy)^2 + abs(vz)^2)^(1/2) + 4*dy*qw*(abs(vx)^2 + abs(vy)^2 + abs(vz)^2)^(1/2)*(qw^2 - qx^2 + qy^2 - qz^2))))/(abs(qw)^2 + abs(qx)^2 + abs(qy)^2 + abs(qz)^2)^(1/2) - (qw*qx*(vx*(2*dx*qx*(2*qw*qz + 2*qx*qy)*(abs(vx)^2 + abs(vy)^2 + abs(vz)^2)^(1/2) + 2*dy*qx*(2*qw*qz - 2*qx*qy)*(abs(vx)^2 + abs(vy)^2 + abs(vz)^2)^(1/2) - 2*dz*qw*(2*qw*qy + 2*qx*qz)*(abs(vx)^2 + abs(vy)^2 + abs(vz)^2)^(1/2) - 2*dz*qz*(2*qw*qx - 2*qy*qz)*(abs(vx)^2 + abs(vy)^2 + abs(vz)^2)^(1/2) + 2*dx*qy*(abs(vx)^2 + abs(vy)^2 + abs(vz)^2)^(1/2)*(qw^2 + qx^2 - qy^2 - qz^2) + 2*dy*qy*(abs(vx)^2 + abs(vy)^2 + abs(vz)^2)^(1/2)*(qw^2 - qx^2 + qy^2 - qz^2)) - vz*(2*dx*qy*(2*qw*qy - 2*qx*qz)*(abs(vx)^2 + abs(vy)^2 + abs(vz)^2)^(1/2) + 2*dy*qx*(2*qw*qx + 2*qy*qz)*(abs(vx)^2 + abs(vy)^2 + abs(vz)^2)^(1/2) - 2*dx*qz*(2*qw*qz + 2*qx*qy)*(abs(vx)^2 + abs(vy)^2 + abs(vz)^2)^(1/2) - 2*dz*qx*(2*qw*qx - 2*qy*qz)*(abs(vx)^2 + abs(vy)^2 + abs(vz)^2)^(1/2) - 2*dy*qw*(abs(vx)^2 + abs(vy)^2 + abs(vz)^2)^(1/2)*(qw^2 - qx^2 + qy^2 - qz^2) + 2*dz*qw*(abs(vx)^2 + abs(vy)^2 + abs(vz)^2)^(1/2)*(qw^2 - qx^2 - qy^2 + qz^2)) + vy*(4*dx*qy*(2*qw*qz + 2*qx*qy)*(abs(vx)^2 + abs(vy)^2 + abs(vz)^2)^(1/2) + 4*dz*qw*(2*qw*qx - 2*qy*qz)*(abs(vx)^2 + abs(vy)^2 + abs(vz)^2)^(1/2) - 4*dy*qx*(abs(vx)^2 + abs(vy)^2 + abs(vz)^2)^(1/2)*(qw^2 - qx^2 + qy^2 - qz^2))))/(abs(qw)^2 + abs(qx)^2 + abs(qy)^2 + abs(qz)^2)^(3/2) + (qw*qz*(vx*(2*dx*qz*(2*qw*qz + 2*qx*qy)*(abs(vx)^2 + abs(vy)^2 + abs(vz)^2)^(1/2) + 2*dz*qx*(2*qw*qx - 2*qy*qz)*(abs(vx)^2 + abs(vy)^2 + abs(vz)^2)^(1/2) - 2*dy*qz*(2*qw*qz - 2*qx*qy)*(abs(vx)^2 + abs(vy)^2 + abs(vz)^2)^(1/2) - 2*dz*qy*(2*qw*qy + 2*qx*qz)*(abs(vx)^2 + abs(vy)^2 + abs(vz)^2)^(1/2) - 2*dx*qw*(abs(vx)^2 + abs(vy)^2 + abs(vz)^2)^(1/2)*(qw^2 + qx^2 - qy^2 - qz^2) + 2*dy*qw*(abs(vx)^2 + abs(vy)^2 + abs(vz)^2)^(1/2)*(qw^2 - qx^2 + qy^2 - qz^2)) + vz*(2*dx*qw*(2*qw*qy - 2*qx*qz)*(abs(vx)^2 + abs(vy)^2 + abs(vz)^2)^(1/2) - 2*dx*qx*(2*qw*qz + 2*qx*qy)*(abs(vx)^2 + abs(vy)^2 + abs(vz)^2)^(1/2) + 2*dy*qz*(2*qw*qx + 2*qy*qz)*(abs(vx)^2 + abs(vy)^2 + abs(vz)^2)^(1/2) + 2*dz*qz*(2*qw*qx - 2*qy*qz)*(abs(vx)^2 + abs(vy)^2 + abs(vz)^2)^(1/2) - 2*dy*qy*(abs(vx)^2 + abs(vy)^2 + abs(vz)^2)^(1/2)*(qw^2 - qx^2 + qy^2 - qz^2) - 2*dz*qy*(abs(vx)^2 + abs(vy)^2 + abs(vz)^2)^(1/2)*(qw^2 - qx^2 - qy^2 + qz^2)) + vy*(4*dz*qy*(2*qw*qx - 2*qy*qz)*(abs(vx)^2 + abs(vy)^2 + abs(vz)^2)^(1/2) - 4*dx*qw*(2*qw*qz + 2*qx*qy)*(abs(vx)^2 + abs(vy)^2 + abs(vz)^2)^(1/2) + 4*dy*qz*(abs(vx)^2 + abs(vy)^2 + abs(vz)^2)^(1/2)*(qw^2 - qx^2 + qy^2 - qz^2))))/(abs(qw)^2 + abs(qx)^2 + abs(qy)^2 + abs(qz)^2)^(3/2) - (qw*qy*(vz*(2*dy*qy*(2*qw*qx + 2*qy*qz)*(abs(vx)^2 + abs(vy)^2 + abs(vz)^2)^(1/2) - 2*dx*qx*(2*qw*qy - 2*qx*qz)*(abs(vx)^2 + abs(vy)^2 + abs(vz)^2)^(1/2) - 2*dx*qw*(2*qw*qz + 2*qx*qy)*(abs(vx)^2 + abs(vy)^2 + abs(vz)^2)^(1/2) + 2*dz*qy*(2*qw*qx - 2*qy*qz)*(abs(vx)^2 + abs(vy)^2 + abs(vz)^2)^(1/2) + 2*dy*qz*(abs(vx)^2 + abs(vy)^2 + abs(vz)^2)^(1/2)*(qw^2 - qx^2 + qy^2 - qz^2) + 2*dz*qz*(abs(vx)^2 + abs(vy)^2 + abs(vz)^2)^(1/2)*(qw^2 - qx^2 - qy^2 + qz^2)) - vx*(2*dx*qy*(2*qw*qz + 2*qx*qy)*(abs(vx)^2 + abs(vy)^2 + abs(vz)^2)^(1/2) + 2*dz*qw*(2*qw*qx - 2*qy*qz)*(abs(vx)^2 + abs(vy)^2 + abs(vz)^2)^(1/2) + 2*dy*qy*(2*qw*qz - 2*qx*qy)*(abs(vx)^2 + abs(vy)^2 + abs(vz)^2)^(1/2) - 2*dz*qz*(2*qw*qy + 2*qx*qz)*(abs(vx)^2 + abs(vy)^2 + abs(vz)^2)^(1/2) - 2*dx*qx*(abs(vx)^2 + abs(vy)^2 + abs(vz)^2)^(1/2)*(qw^2 + qx^2 - qy^2 - qz^2) - 2*dy*qx*(abs(vx)^2 + abs(vy)^2 + abs(vz)^2)^(1/2)*(qw^2 - qx^2 + qy^2 - qz^2)) + vy*(4*dx*qx*(2*qw*qz + 2*qx*qy)*(abs(vx)^2 + abs(vy)^2 + abs(vz)^2)^(1/2) - 4*dz*qz*(2*qw*qx - 2*qy*qz)*(abs(vx)^2 + abs(vy)^2 + abs(vz)^2)^(1/2) + 4*dy*qy*(abs(vx)^2 + abs(vy)^2 + abs(vz)^2)^(1/2)*(qw^2 - qx^2 + qy^2 - qz^2))))/(abs(qw)^2 + abs(qx)^2 + abs(qy)^2 + abs(qz)^2)^(3/2), (qw*qx*(vx*(2*dy*qw*(2*qw*qz - 2*qx*qy)*(abs(vx)^2 + abs(vy)^2 + abs(vz)^2)^(1/2) - 2*dx*qw*(2*qw*qz + 2*qx*qy)*(abs(vx)^2 + abs(vy)^2 + abs(vz)^2)^(1/2) + 2*dz*qx*(2*qw*qy + 2*qx*qz)*(abs(vx)^2 + abs(vy)^2 + abs(vz)^2)^(1/2) + 2*dz*qy*(2*qw*qx - 2*qy*qz)*(abs(vx)^2 + abs(vy)^2 + abs(vz)^2)^(1/2) - 2*dx*qz*(abs(vx)^2 + abs(vy)^2 + abs(vz)^2)^(1/2)*(qw^2 + qx^2 - qy^2 - qz^2) + 2*dy*qz*(abs(vx)^2 + abs(vy)^2 + abs(vz)^2)^(1/2)*(qw^2 - qx^2 + qy^2 - qz^2)) + vz*(2*dx*qy*(2*qw*qz + 2*qx*qy)*(abs(vx)^2 + abs(vy)^2 + abs(vz)^2)^(1/2) - 2*dy*qw*(2*qw*qx + 2*qy*qz)*(abs(vx)^2 + abs(vy)^2 + abs(vz)^2)^(1/2) + 2*dz*qw*(2*qw*qx - 2*qy*qz)*(abs(vx)^2 + abs(vy)^2 + abs(vz)^2)^(1/2) + 2*dx*qz*(2*qw*qy - 2*qx*qz)*(abs(vx)^2 + abs(vy)^2 + abs(vz)^2)^(1/2) - 2*dy*qx*(abs(vx)^2 + abs(vy)^2 + abs(vz)^2)^(1/2)*(qw^2 - qx^2 + qy^2 - qz^2) + 2*dz*qx*(abs(vx)^2 + abs(vy)^2 + abs(vz)^2)^(1/2)*(qw^2 - qx^2 - qy^2 + qz^2)) - vy*(4*dx*qz*(2*qw*qz + 2*qx*qy)*(abs(vx)^2 + abs(vy)^2 + abs(vz)^2)^(1/2) + 4*dz*qx*(2*qw*qx - 2*qy*qz)*(abs(vx)^2 + abs(vy)^2 + abs(vz)^2)^(1/2) + 4*dy*qw*(abs(vx)^2 + abs(vy)^2 + abs(vz)^2)^(1/2)*(qw^2 - qx^2 + qy^2 - qz^2))))/(abs(qw)^2 + abs(qx)^2 + abs(qy)^2 + abs(qz)^2)^(3/2) - ((qx^2/(abs(qw)^2 + abs(qx)^2 + abs(qy)^2 + abs(qz)^2) - 1)*(vx*(2*dx*qx*(2*qw*qz + 2*qx*qy)*(abs(vx)^2 + abs(vy)^2 + abs(vz)^2)^(1/2) + 2*dy*qx*(2*qw*qz - 2*qx*qy)*(abs(vx)^2 + abs(vy)^2 + abs(vz)^2)^(1/2) - 2*dz*qw*(2*qw*qy + 2*qx*qz)*(abs(vx)^2 + abs(vy)^2 + abs(vz)^2)^(1/2) - 2*dz*qz*(2*qw*qx - 2*qy*qz)*(abs(vx)^2 + abs(vy)^2 + abs(vz)^2)^(1/2) + 2*dx*qy*(abs(vx)^2 + abs(vy)^2 + abs(vz)^2)^(1/2)*(qw^2 + qx^2 - qy^2 - qz^2) + 2*dy*qy*(abs(vx)^2 + abs(vy)^2 + abs(vz)^2)^(1/2)*(qw^2 - qx^2 + qy^2 - qz^2)) - vz*(2*dx*qy*(2*qw*qy - 2*qx*qz)*(abs(vx)^2 + abs(vy)^2 + abs(vz)^2)^(1/2) + 2*dy*qx*(2*qw*qx + 2*qy*qz)*(abs(vx)^2 + abs(vy)^2 + abs(vz)^2)^(1/2) - 2*dx*qz*(2*qw*qz + 2*qx*qy)*(abs(vx)^2 + abs(vy)^2 + abs(vz)^2)^(1/2) - 2*dz*qx*(2*qw*qx - 2*qy*qz)*(abs(vx)^2 + abs(vy)^2 + abs(vz)^2)^(1/2) - 2*dy*qw*(abs(vx)^2 + abs(vy)^2 + abs(vz)^2)^(1/2)*(qw^2 - qx^2 + qy^2 - qz^2) + 2*dz*qw*(abs(vx)^2 + abs(vy)^2 + abs(vz)^2)^(1/2)*(qw^2 - qx^2 - qy^2 + qz^2)) + vy*(4*dx*qy*(2*qw*qz + 2*qx*qy)*(abs(vx)^2 + abs(vy)^2 + abs(vz)^2)^(1/2) + 4*dz*qw*(2*qw*qx - 2*qy*qz)*(abs(vx)^2 + abs(vy)^2 + abs(vz)^2)^(1/2) - 4*dy*qx*(abs(vx)^2 + abs(vy)^2 + abs(vz)^2)^(1/2)*(qw^2 - qx^2 + qy^2 - qz^2))))/(abs(qw)^2 + abs(qx)^2 + abs(qy)^2 + abs(qz)^2)^(1/2) + (qx*qz*(vx*(2*dx*qz*(2*qw*qz + 2*qx*qy)*(abs(vx)^2 + abs(vy)^2 + abs(vz)^2)^(1/2) + 2*dz*qx*(2*qw*qx - 2*qy*qz)*(abs(vx)^2 + abs(vy)^2 + abs(vz)^2)^(1/2) - 2*dy*qz*(2*qw*qz - 2*qx*qy)*(abs(vx)^2 + abs(vy)^2 + abs(vz)^2)^(1/2) - 2*dz*qy*(2*qw*qy + 2*qx*qz)*(abs(vx)^2 + abs(vy)^2 + abs(vz)^2)^(1/2) - 2*dx*qw*(abs(vx)^2 + abs(vy)^2 + abs(vz)^2)^(1/2)*(qw^2 + qx^2 - qy^2 - qz^2) + 2*dy*qw*(abs(vx)^2 + abs(vy)^2 + abs(vz)^2)^(1/2)*(qw^2 - qx^2 + qy^2 - qz^2)) + vz*(2*dx*qw*(2*qw*qy - 2*qx*qz)*(abs(vx)^2 + abs(vy)^2 + abs(vz)^2)^(1/2) - 2*dx*qx*(2*qw*qz + 2*qx*qy)*(abs(vx)^2 + abs(vy)^2 + abs(vz)^2)^(1/2) + 2*dy*qz*(2*qw*qx + 2*qy*qz)*(abs(vx)^2 + abs(vy)^2 + abs(vz)^2)^(1/2) + 2*dz*qz*(2*qw*qx - 2*qy*qz)*(abs(vx)^2 + abs(vy)^2 + abs(vz)^2)^(1/2) - 2*dy*qy*(abs(vx)^2 + abs(vy)^2 + abs(vz)^2)^(1/2)*(qw^2 - qx^2 + qy^2 - qz^2) - 2*dz*qy*(abs(vx)^2 + abs(vy)^2 + abs(vz)^2)^(1/2)*(qw^2 - qx^2 - qy^2 + qz^2)) + vy*(4*dz*qy*(2*qw*qx - 2*qy*qz)*(abs(vx)^2 + abs(vy)^2 + abs(vz)^2)^(1/2) - 4*dx*qw*(2*qw*qz + 2*qx*qy)*(abs(vx)^2 + abs(vy)^2 + abs(vz)^2)^(1/2) + 4*dy*qz*(abs(vx)^2 + abs(vy)^2 + abs(vz)^2)^(1/2)*(qw^2 - qx^2 + qy^2 - qz^2))))/(abs(qw)^2 + abs(qx)^2 + abs(qy)^2 + abs(qz)^2)^(3/2) - (qx*qy*(vz*(2*dy*qy*(2*qw*qx + 2*qy*qz)*(abs(vx)^2 + abs(vy)^2 + abs(vz)^2)^(1/2) - 2*dx*qx*(2*qw*qy - 2*qx*qz)*(abs(vx)^2 + abs(vy)^2 + abs(vz)^2)^(1/2) - 2*dx*qw*(2*qw*qz + 2*qx*qy)*(abs(vx)^2 + abs(vy)^2 + abs(vz)^2)^(1/2) + 2*dz*qy*(2*qw*qx - 2*qy*qz)*(abs(vx)^2 + abs(vy)^2 + abs(vz)^2)^(1/2) + 2*dy*qz*(abs(vx)^2 + abs(vy)^2 + abs(vz)^2)^(1/2)*(qw^2 - qx^2 + qy^2 - qz^2) + 2*dz*qz*(abs(vx)^2 + abs(vy)^2 + abs(vz)^2)^(1/2)*(qw^2 - qx^2 - qy^2 + qz^2)) - vx*(2*dx*qy*(2*qw*qz + 2*qx*qy)*(abs(vx)^2 + abs(vy)^2 + abs(vz)^2)^(1/2) + 2*dz*qw*(2*qw*qx - 2*qy*qz)*(abs(vx)^2 + abs(vy)^2 + abs(vz)^2)^(1/2) + 2*dy*qy*(2*qw*qz - 2*qx*qy)*(abs(vx)^2 + abs(vy)^2 + abs(vz)^2)^(1/2) - 2*dz*qz*(2*qw*qy + 2*qx*qz)*(abs(vx)^2 + abs(vy)^2 + abs(vz)^2)^(1/2) - 2*dx*qx*(abs(vx)^2 + abs(vy)^2 + abs(vz)^2)^(1/2)*(qw^2 + qx^2 - qy^2 - qz^2) - 2*dy*qx*(abs(vx)^2 + abs(vy)^2 + abs(vz)^2)^(1/2)*(qw^2 - qx^2 + qy^2 - qz^2)) + vy*(4*dx*qx*(2*qw*qz + 2*qx*qy)*(abs(vx)^2 + abs(vy)^2 + abs(vz)^2)^(1/2) - 4*dz*qz*(2*qw*qx - 2*qy*qz)*(abs(vx)^2 + abs(vy)^2 + abs(vz)^2)^(1/2) + 4*dy*qy*(abs(vx)^2 + abs(vy)^2 + abs(vz)^2)^(1/2)*(qw^2 - qx^2 + qy^2 - qz^2))))/(abs(qw)^2 + abs(qx)^2 + abs(qy)^2 + abs(qz)^2)^(3/2), (qw*qy*(vx*(2*dy*qw*(2*qw*qz - 2*qx*qy)*(abs(vx)^2 + abs(vy)^2 + abs(vz)^2)^(1/2) - 2*dx*qw*(2*qw*qz + 2*qx*qy)*(abs(vx)^2 + abs(vy)^2 + abs(vz)^2)^(1/2) + 2*dz*qx*(2*qw*qy + 2*qx*qz)*(abs(vx)^2 + abs(vy)^2 + abs(vz)^2)^(1/2) + 2*dz*qy*(2*qw*qx - 2*qy*qz)*(abs(vx)^2 + abs(vy)^2 + abs(vz)^2)^(1/2) - 2*dx*qz*(abs(vx)^2 + abs(vy)^2 + abs(vz)^2)^(1/2)*(qw^2 + qx^2 - qy^2 - qz^2) + 2*dy*qz*(abs(vx)^2 + abs(vy)^2 + abs(vz)^2)^(1/2)*(qw^2 - qx^2 + qy^2 - qz^2)) + vz*(2*dx*qy*(2*qw*qz + 2*qx*qy)*(abs(vx)^2 + abs(vy)^2 + abs(vz)^2)^(1/2) - 2*dy*qw*(2*qw*qx + 2*qy*qz)*(abs(vx)^2 + abs(vy)^2 + abs(vz)^2)^(1/2) + 2*dz*qw*(2*qw*qx - 2*qy*qz)*(abs(vx)^2 + abs(vy)^2 + abs(vz)^2)^(1/2) + 2*dx*qz*(2*qw*qy - 2*qx*qz)*(abs(vx)^2 + abs(vy)^2 + abs(vz)^2)^(1/2) - 2*dy*qx*(abs(vx)^2 + abs(vy)^2 + abs(vz)^2)^(1/2)*(qw^2 - qx^2 + qy^2 - qz^2) + 2*dz*qx*(abs(vx)^2 + abs(vy)^2 + abs(vz)^2)^(1/2)*(qw^2 - qx^2 - qy^2 + qz^2)) - vy*(4*dx*qz*(2*qw*qz + 2*qx*qy)*(abs(vx)^2 + abs(vy)^2 + abs(vz)^2)^(1/2) + 4*dz*qx*(2*qw*qx - 2*qy*qz)*(abs(vx)^2 + abs(vy)^2 + abs(vz)^2)^(1/2) + 4*dy*qw*(abs(vx)^2 + abs(vy)^2 + abs(vz)^2)^(1/2)*(qw^2 - qx^2 + qy^2 - qz^2))))/(abs(qw)^2 + abs(qx)^2 + abs(qy)^2 + abs(qz)^2)^(3/2) - ((qy^2/(abs(qw)^2 + abs(qx)^2 + abs(qy)^2 + abs(qz)^2) - 1)*(vz*(2*dy*qy*(2*qw*qx + 2*qy*qz)*(abs(vx)^2 + abs(vy)^2 + abs(vz)^2)^(1/2) - 2*dx*qx*(2*qw*qy - 2*qx*qz)*(abs(vx)^2 + abs(vy)^2 + abs(vz)^2)^(1/2) - 2*dx*qw*(2*qw*qz + 2*qx*qy)*(abs(vx)^2 + abs(vy)^2 + abs(vz)^2)^(1/2) + 2*dz*qy*(2*qw*qx - 2*qy*qz)*(abs(vx)^2 + abs(vy)^2 + abs(vz)^2)^(1/2) + 2*dy*qz*(abs(vx)^2 + abs(vy)^2 + abs(vz)^2)^(1/2)*(qw^2 - qx^2 + qy^2 - qz^2) + 2*dz*qz*(abs(vx)^2 + abs(vy)^2 + abs(vz)^2)^(1/2)*(qw^2 - qx^2 - qy^2 + qz^2)) - vx*(2*dx*qy*(2*qw*qz + 2*qx*qy)*(abs(vx)^2 + abs(vy)^2 + abs(vz)^2)^(1/2) + 2*dz*qw*(2*qw*qx - 2*qy*qz)*(abs(vx)^2 + abs(vy)^2 + abs(vz)^2)^(1/2) + 2*dy*qy*(2*qw*qz - 2*qx*qy)*(abs(vx)^2 + abs(vy)^2 + abs(vz)^2)^(1/2) - 2*dz*qz*(2*qw*qy + 2*qx*qz)*(abs(vx)^2 + abs(vy)^2 + abs(vz)^2)^(1/2) - 2*dx*qx*(abs(vx)^2 + abs(vy)^2 + abs(vz)^2)^(1/2)*(qw^2 + qx^2 - qy^2 - qz^2) - 2*dy*qx*(abs(vx)^2 + abs(vy)^2 + abs(vz)^2)^(1/2)*(qw^2 - qx^2 + qy^2 - qz^2)) + vy*(4*dx*qx*(2*qw*qz + 2*qx*qy)*(abs(vx)^2 + abs(vy)^2 + abs(vz)^2)^(1/2) - 4*dz*qz*(2*qw*qx - 2*qy*qz)*(abs(vx)^2 + abs(vy)^2 + abs(vz)^2)^(1/2) + 4*dy*qy*(abs(vx)^2 + abs(vy)^2 + abs(vz)^2)^(1/2)*(qw^2 - qx^2 + qy^2 - qz^2))))/(abs(qw)^2 + abs(qx)^2 + abs(qy)^2 + abs(qz)^2)^(1/2) - (qx*qy*(vx*(2*dx*qx*(2*qw*qz + 2*qx*qy)*(abs(vx)^2 + abs(vy)^2 + abs(vz)^2)^(1/2) + 2*dy*qx*(2*qw*qz - 2*qx*qy)*(abs(vx)^2 + abs(vy)^2 + abs(vz)^2)^(1/2) - 2*dz*qw*(2*qw*qy + 2*qx*qz)*(abs(vx)^2 + abs(vy)^2 + abs(vz)^2)^(1/2) - 2*dz*qz*(2*qw*qx - 2*qy*qz)*(abs(vx)^2 + abs(vy)^2 + abs(vz)^2)^(1/2) + 2*dx*qy*(abs(vx)^2 + abs(vy)^2 + abs(vz)^2)^(1/2)*(qw^2 + qx^2 - qy^2 - qz^2) + 2*dy*qy*(abs(vx)^2 + abs(vy)^2 + abs(vz)^2)^(1/2)*(qw^2 - qx^2 + qy^2 - qz^2)) - vz*(2*dx*qy*(2*qw*qy - 2*qx*qz)*(abs(vx)^2 + abs(vy)^2 + abs(vz)^2)^(1/2) + 2*dy*qx*(2*qw*qx + 2*qy*qz)*(abs(vx)^2 + abs(vy)^2 + abs(vz)^2)^(1/2) - 2*dx*qz*(2*qw*qz + 2*qx*qy)*(abs(vx)^2 + abs(vy)^2 + abs(vz)^2)^(1/2) - 2*dz*qx*(2*qw*qx - 2*qy*qz)*(abs(vx)^2 + abs(vy)^2 + abs(vz)^2)^(1/2) - 2*dy*qw*(abs(vx)^2 + abs(vy)^2 + abs(vz)^2)^(1/2)*(qw^2 - qx^2 + qy^2 - qz^2) + 2*dz*qw*(abs(vx)^2 + abs(vy)^2 + abs(vz)^2)^(1/2)*(qw^2 - qx^2 - qy^2 + qz^2)) + vy*(4*dx*qy*(2*qw*qz + 2*qx*qy)*(abs(vx)^2 + abs(vy)^2 + abs(vz)^2)^(1/2) + 4*dz*qw*(2*qw*qx - 2*qy*qz)*(abs(vx)^2 + abs(vy)^2 + abs(vz)^2)^(1/2) - 4*dy*qx*(abs(vx)^2 + abs(vy)^2 + abs(vz)^2)^(1/2)*(qw^2 - qx^2 + qy^2 - qz^2))))/(abs(qw)^2 + abs(qx)^2 + abs(qy)^2 + abs(qz)^2)^(3/2) + (qy*qz*(vx*(2*dx*qz*(2*qw*qz + 2*qx*qy)*(abs(vx)^2 + abs(vy)^2 + abs(vz)^2)^(1/2) + 2*dz*qx*(2*qw*qx - 2*qy*qz)*(abs(vx)^2 + abs(vy)^2 + abs(vz)^2)^(1/2) - 2*dy*qz*(2*qw*qz - 2*qx*qy)*(abs(vx)^2 + abs(vy)^2 + abs(vz)^2)^(1/2) - 2*dz*qy*(2*qw*qy + 2*qx*qz)*(abs(vx)^2 + abs(vy)^2 + abs(vz)^2)^(1/2) - 2*dx*qw*(abs(vx)^2 + abs(vy)^2 + abs(vz)^2)^(1/2)*(qw^2 + qx^2 - qy^2 - qz^2) + 2*dy*qw*(abs(vx)^2 + abs(vy)^2 + abs(vz)^2)^(1/2)*(qw^2 - qx^2 + qy^2 - qz^2)) + vz*(2*dx*qw*(2*qw*qy - 2*qx*qz)*(abs(vx)^2 + abs(vy)^2 + abs(vz)^2)^(1/2) - 2*dx*qx*(2*qw*qz + 2*qx*qy)*(abs(vx)^2 + abs(vy)^2 + abs(vz)^2)^(1/2) + 2*dy*qz*(2*qw*qx + 2*qy*qz)*(abs(vx)^2 + abs(vy)^2 + abs(vz)^2)^(1/2) + 2*dz*qz*(2*qw*qx - 2*qy*qz)*(abs(vx)^2 + abs(vy)^2 + abs(vz)^2)^(1/2) - 2*dy*qy*(abs(vx)^2 + abs(vy)^2 + abs(vz)^2)^(1/2)*(qw^2 - qx^2 + qy^2 - qz^2) - 2*dz*qy*(abs(vx)^2 + abs(vy)^2 + abs(vz)^2)^(1/2)*(qw^2 - qx^2 - qy^2 + qz^2)) + vy*(4*dz*qy*(2*qw*qx - 2*qy*qz)*(abs(vx)^2 + abs(vy)^2 + abs(vz)^2)^(1/2) - 4*dx*qw*(2*qw*qz + 2*qx*qy)*(abs(vx)^2 + abs(vy)^2 + abs(vz)^2)^(1/2) + 4*dy*qz*(abs(vx)^2 + abs(vy)^2 + abs(vz)^2)^(1/2)*(qw^2 - qx^2 + qy^2 - qz^2))))/(abs(qw)^2 + abs(qx)^2 + abs(qy)^2 + abs(qz)^2)^(3/2), ((qz^2/(abs(qw)^2 + abs(qx)^2 + abs(qy)^2 + abs(qz)^2) - 1)*(vx*(2*dx*qz*(2*qw*qz + 2*qx*qy)*(abs(vx)^2 + abs(vy)^2 + abs(vz)^2)^(1/2) + 2*dz*qx*(2*qw*qx - 2*qy*qz)*(abs(vx)^2 + abs(vy)^2 + abs(vz)^2)^(1/2) - 2*dy*qz*(2*qw*qz - 2*qx*qy)*(abs(vx)^2 + abs(vy)^2 + abs(vz)^2)^(1/2) - 2*dz*qy*(2*qw*qy + 2*qx*qz)*(abs(vx)^2 + abs(vy)^2 + abs(vz)^2)^(1/2) - 2*dx*qw*(abs(vx)^2 + abs(vy)^2 + abs(vz)^2)^(1/2)*(qw^2 + qx^2 - qy^2 - qz^2) + 2*dy*qw*(abs(vx)^2 + abs(vy)^2 + abs(vz)^2)^(1/2)*(qw^2 - qx^2 + qy^2 - qz^2)) + vz*(2*dx*qw*(2*qw*qy - 2*qx*qz)*(abs(vx)^2 + abs(vy)^2 + abs(vz)^2)^(1/2) - 2*dx*qx*(2*qw*qz + 2*qx*qy)*(abs(vx)^2 + abs(vy)^2 + abs(vz)^2)^(1/2) + 2*dy*qz*(2*qw*qx + 2*qy*qz)*(abs(vx)^2 + abs(vy)^2 + abs(vz)^2)^(1/2) + 2*dz*qz*(2*qw*qx - 2*qy*qz)*(abs(vx)^2 + abs(vy)^2 + abs(vz)^2)^(1/2) - 2*dy*qy*(abs(vx)^2 + abs(vy)^2 + abs(vz)^2)^(1/2)*(qw^2 - qx^2 + qy^2 - qz^2) - 2*dz*qy*(abs(vx)^2 + abs(vy)^2 + abs(vz)^2)^(1/2)*(qw^2 - qx^2 - qy^2 + qz^2)) + vy*(4*dz*qy*(2*qw*qx - 2*qy*qz)*(abs(vx)^2 + abs(vy)^2 + abs(vz)^2)^(1/2) - 4*dx*qw*(2*qw*qz + 2*qx*qy)*(abs(vx)^2 + abs(vy)^2 + abs(vz)^2)^(1/2) + 4*dy*qz*(abs(vx)^2 + abs(vy)^2 + abs(vz)^2)^(1/2)*(qw^2 - qx^2 + qy^2 - qz^2))))/(abs(qw)^2 + abs(qx)^2 + abs(qy)^2 + abs(qz)^2)^(1/2) + (qw*qz*(vx*(2*dy*qw*(2*qw*qz - 2*qx*qy)*(abs(vx)^2 + abs(vy)^2 + abs(vz)^2)^(1/2) - 2*dx*qw*(2*qw*qz + 2*qx*qy)*(abs(vx)^2 + abs(vy)^2 + abs(vz)^2)^(1/2) + 2*dz*qx*(2*qw*qy + 2*qx*qz)*(abs(vx)^2 + abs(vy)^2 + abs(vz)^2)^(1/2) + 2*dz*qy*(2*qw*qx - 2*qy*qz)*(abs(vx)^2 + abs(vy)^2 + abs(vz)^2)^(1/2) - 2*dx*qz*(abs(vx)^2 + abs(vy)^2 + abs(vz)^2)^(1/2)*(qw^2 + qx^2 - qy^2 - qz^2) + 2*dy*qz*(abs(vx)^2 + abs(vy)^2 + abs(vz)^2)^(1/2)*(qw^2 - qx^2 + qy^2 - qz^2)) + vz*(2*dx*qy*(2*qw*qz + 2*qx*qy)*(abs(vx)^2 + abs(vy)^2 + abs(vz)^2)^(1/2) - 2*dy*qw*(2*qw*qx + 2*qy*qz)*(abs(vx)^2 + abs(vy)^2 + abs(vz)^2)^(1/2) + 2*dz*qw*(2*qw*qx - 2*qy*qz)*(abs(vx)^2 + abs(vy)^2 + abs(vz)^2)^(1/2) + 2*dx*qz*(2*qw*qy - 2*qx*qz)*(abs(vx)^2 + abs(vy)^2 + abs(vz)^2)^(1/2) - 2*dy*qx*(abs(vx)^2 + abs(vy)^2 + abs(vz)^2)^(1/2)*(qw^2 - qx^2 + qy^2 - qz^2) + 2*dz*qx*(abs(vx)^2 + abs(vy)^2 + abs(vz)^2)^(1/2)*(qw^2 - qx^2 - qy^2 + qz^2)) - vy*(4*dx*qz*(2*qw*qz + 2*qx*qy)*(abs(vx)^2 + abs(vy)^2 + abs(vz)^2)^(1/2) + 4*dz*qx*(2*qw*qx - 2*qy*qz)*(abs(vx)^2 + abs(vy)^2 + abs(vz)^2)^(1/2) + 4*dy*qw*(abs(vx)^2 + abs(vy)^2 + abs(vz)^2)^(1/2)*(qw^2 - qx^2 + qy^2 - qz^2))))/(abs(qw)^2 + abs(qx)^2 + abs(qy)^2 + abs(qz)^2)^(3/2) - (qx*qz*(vx*(2*dx*qx*(2*qw*qz + 2*qx*qy)*(abs(vx)^2 + abs(vy)^2 + abs(vz)^2)^(1/2) + 2*dy*qx*(2*qw*qz - 2*qx*qy)*(abs(vx)^2 + abs(vy)^2 + abs(vz)^2)^(1/2) - 2*dz*qw*(2*qw*qy + 2*qx*qz)*(abs(vx)^2 + abs(vy)^2 + abs(vz)^2)^(1/2) - 2*dz*qz*(2*qw*qx - 2*qy*qz)*(abs(vx)^2 + abs(vy)^2 + abs(vz)^2)^(1/2) + 2*dx*qy*(abs(vx)^2 + abs(vy)^2 + abs(vz)^2)^(1/2)*(qw^2 + qx^2 - qy^2 - qz^2) + 2*dy*qy*(abs(vx)^2 + abs(vy)^2 + abs(vz)^2)^(1/2)*(qw^2 - qx^2 + qy^2 - qz^2)) - vz*(2*dx*qy*(2*qw*qy - 2*qx*qz)*(abs(vx)^2 + abs(vy)^2 + abs(vz)^2)^(1/2) + 2*dy*qx*(2*qw*qx + 2*qy*qz)*(abs(vx)^2 + abs(vy)^2 + abs(vz)^2)^(1/2) - 2*dx*qz*(2*qw*qz + 2*qx*qy)*(abs(vx)^2 + abs(vy)^2 + abs(vz)^2)^(1/2) - 2*dz*qx*(2*qw*qx - 2*qy*qz)*(abs(vx)^2 + abs(vy)^2 + abs(vz)^2)^(1/2) - 2*dy*qw*(abs(vx)^2 + abs(vy)^2 + abs(vz)^2)^(1/2)*(qw^2 - qx^2 + qy^2 - qz^2) + 2*dz*qw*(abs(vx)^2 + abs(vy)^2 + abs(vz)^2)^(1/2)*(qw^2 - qx^2 - qy^2 + qz^2)) + vy*(4*dx*qy*(2*qw*qz + 2*qx*qy)*(abs(vx)^2 + abs(vy)^2 + abs(vz)^2)^(1/2) + 4*dz*qw*(2*qw*qx - 2*qy*qz)*(abs(vx)^2 + abs(vy)^2 + abs(vz)^2)^(1/2) - 4*dy*qx*(abs(vx)^2 + abs(vy)^2 + abs(vz)^2)^(1/2)*(qw^2 - qx^2 + qy^2 - qz^2))))/(abs(qw)^2 + abs(qx)^2 + abs(qy)^2 + abs(qz)^2)^(3/2) - (qy*qz*(vz*(2*dy*qy*(2*qw*qx + 2*qy*qz)*(abs(vx)^2 + abs(vy)^2 + abs(vz)^2)^(1/2) - 2*dx*qx*(2*qw*qy - 2*qx*qz)*(abs(vx)^2 + abs(vy)^2 + abs(vz)^2)^(1/2) - 2*dx*qw*(2*qw*qz + 2*qx*qy)*(abs(vx)^2 + abs(vy)^2 + abs(vz)^2)^(1/2) + 2*dz*qy*(2*qw*qx - 2*qy*qz)*(abs(vx)^2 + abs(vy)^2 + abs(vz)^2)^(1/2) + 2*dy*qz*(abs(vx)^2 + abs(vy)^2 + abs(vz)^2)^(1/2)*(qw^2 - qx^2 + qy^2 - qz^2) + 2*dz*qz*(abs(vx)^2 + abs(vy)^2 + abs(vz)^2)^(1/2)*(qw^2 - qx^2 - qy^2 + qz^2)) - vx*(2*dx*qy*(2*qw*qz + 2*qx*qy)*(abs(vx)^2 + abs(vy)^2 + abs(vz)^2)^(1/2) + 2*dz*qw*(2*qw*qx - 2*qy*qz)*(abs(vx)^2 + abs(vy)^2 + abs(vz)^2)^(1/2) + 2*dy*qy*(2*qw*qz - 2*qx*qy)*(abs(vx)^2 + abs(vy)^2 + abs(vz)^2)^(1/2) - 2*dz*qz*(2*qw*qy + 2*qx*qz)*(abs(vx)^2 + abs(vy)^2 + abs(vz)^2)^(1/2) - 2*dx*qx*(abs(vx)^2 + abs(vy)^2 + abs(vz)^2)^(1/2)*(qw^2 + qx^2 - qy^2 - qz^2) - 2*dy*qx*(abs(vx)^2 + abs(vy)^2 + abs(vz)^2)^(1/2)*(qw^2 - qx^2 + qy^2 - qz^2)) + vy*(4*dx*qx*(2*qw*qz + 2*qx*qy)*(abs(vx)^2 + abs(vy)^2 + abs(vz)^2)^(1/2) - 4*dz*qz*(2*qw*qx - 2*qy*qz)*(abs(vx)^2 + abs(vy)^2 + abs(vz)^2)^(1/2) + 4*dy*qy*(abs(vx)^2 + abs(vy)^2 + abs(vz)^2)^(1/2)*(qw^2 - qx^2 + qy^2 - qz^2))))/(abs(qw)^2 + abs(qx)^2 + abs(qy)^2 + abs(qz)^2)^(3/2);
%  ((qw^2/(abs(qw)^2 + abs(qx)^2 + abs(qy)^2 + abs(qz)^2) - 1)*(vx*(2*dx*qw*(2*qw*qy - 2*qx*qz)*(abs(vx)^2 + abs(vy)^2 + abs(vz)^2)^(1/2) + 2*dy*qx*(2*qw*qz - 2*qx*qy)*(abs(vx)^2 + abs(vy)^2 + abs(vz)^2)^(1/2) - 2*dz*qw*(2*qw*qy + 2*qx*qz)*(abs(vx)^2 + abs(vy)^2 + abs(vz)^2)^(1/2) + 2*dy*qz*(2*qw*qx + 2*qy*qz)*(abs(vx)^2 + abs(vy)^2 + abs(vz)^2)^(1/2) + 2*dx*qy*(abs(vx)^2 + abs(vy)^2 + abs(vz)^2)^(1/2)*(qw^2 + qx^2 - qy^2 - qz^2) - 2*dz*qy*(abs(vx)^2 + abs(vy)^2 + abs(vz)^2)^(1/2)*(qw^2 - qx^2 - qy^2 + qz^2)) + vy*(2*dx*qy*(2*qw*qz + 2*qx*qy)*(abs(vx)^2 + abs(vy)^2 + abs(vz)^2)^(1/2) - 2*dy*qw*(2*qw*qx + 2*qy*qz)*(abs(vx)^2 + abs(vy)^2 + abs(vz)^2)^(1/2) + 2*dz*qw*(2*qw*qx - 2*qy*qz)*(abs(vx)^2 + abs(vy)^2 + abs(vz)^2)^(1/2) + 2*dx*qz*(2*qw*qy - 2*qx*qz)*(abs(vx)^2 + abs(vy)^2 + abs(vz)^2)^(1/2) - 2*dy*qx*(abs(vx)^2 + abs(vy)^2 + abs(vz)^2)^(1/2)*(qw^2 - qx^2 + qy^2 - qz^2) + 2*dz*qx*(abs(vx)^2 + abs(vy)^2 + abs(vz)^2)^(1/2)*(qw^2 - qx^2 - qy^2 + qz^2)) - vz*(4*dx*qy*(2*qw*qy - 2*qx*qz)*(abs(vx)^2 + abs(vy)^2 + abs(vz)^2)^(1/2) + 4*dy*qx*(2*qw*qx + 2*qy*qz)*(abs(vx)^2 + abs(vy)^2 + abs(vz)^2)^(1/2) + 4*dz*qw*(abs(vx)^2 + abs(vy)^2 + abs(vz)^2)^(1/2)*(qw^2 - qx^2 - qy^2 + qz^2))))/(abs(qw)^2 + abs(qx)^2 + abs(qy)^2 + abs(qz)^2)^(1/2) + (qw*qx*(vy*(2*dx*qy*(2*qw*qy - 2*qx*qz)*(abs(vx)^2 + abs(vy)^2 + abs(vz)^2)^(1/2) + 2*dy*qx*(2*qw*qx + 2*qy*qz)*(abs(vx)^2 + abs(vy)^2 + abs(vz)^2)^(1/2) - 2*dx*qz*(2*qw*qz + 2*qx*qy)*(abs(vx)^2 + abs(vy)^2 + abs(vz)^2)^(1/2) - 2*dz*qx*(2*qw*qx - 2*qy*qz)*(abs(vx)^2 + abs(vy)^2 + abs(vz)^2)^(1/2) - 2*dy*qw*(abs(vx)^2 + abs(vy)^2 + abs(vz)^2)^(1/2)*(qw^2 - qx^2 + qy^2 - qz^2) + 2*dz*qw*(abs(vx)^2 + abs(vy)^2 + abs(vz)^2)^(1/2)*(qw^2 - qx^2 - qy^2 + qz^2)) + vx*(2*dx*qx*(2*qw*qy - 2*qx*qz)*(abs(vx)^2 + abs(vy)^2 + abs(vz)^2)^(1/2) + 2*dy*qw*(2*qw*qz - 2*qx*qy)*(abs(vx)^2 + abs(vy)^2 + abs(vz)^2)^(1/2) - 2*dy*qy*(2*qw*qx + 2*qy*qz)*(abs(vx)^2 + abs(vy)^2 + abs(vz)^2)^(1/2) + 2*dz*qx*(2*qw*qy + 2*qx*qz)*(abs(vx)^2 + abs(vy)^2 + abs(vz)^2)^(1/2) - 2*dx*qz*(abs(vx)^2 + abs(vy)^2 + abs(vz)^2)^(1/2)*(qw^2 + qx^2 - qy^2 - qz^2) - 2*dz*qz*(abs(vx)^2 + abs(vy)^2 + abs(vz)^2)^(1/2)*(qw^2 - qx^2 - qy^2 + qz^2)) + vz*(4*dx*qz*(2*qw*qy - 2*qx*qz)*(abs(vx)^2 + abs(vy)^2 + abs(vz)^2)^(1/2) - 4*dy*qw*(2*qw*qx + 2*qy*qz)*(abs(vx)^2 + abs(vy)^2 + abs(vz)^2)^(1/2) + 4*dz*qx*(abs(vx)^2 + abs(vy)^2 + abs(vz)^2)^(1/2)*(qw^2 - qx^2 - qy^2 + qz^2))))/(abs(qw)^2 + abs(qx)^2 + abs(qy)^2 + abs(qz)^2)^(3/2) - (qw*qy*(vx*(2*dx*qy*(2*qw*qy - 2*qx*qz)*(abs(vx)^2 + abs(vy)^2 + abs(vz)^2)^(1/2) + 2*dy*qx*(2*qw*qx + 2*qy*qz)*(abs(vx)^2 + abs(vy)^2 + abs(vz)^2)^(1/2) - 2*dy*qz*(2*qw*qz - 2*qx*qy)*(abs(vx)^2 + abs(vy)^2 + abs(vz)^2)^(1/2) - 2*dz*qy*(2*qw*qy + 2*qx*qz)*(abs(vx)^2 + abs(vy)^2 + abs(vz)^2)^(1/2) - 2*dx*qw*(abs(vx)^2 + abs(vy)^2 + abs(vz)^2)^(1/2)*(qw^2 + qx^2 - qy^2 - qz^2) + 2*dz*qw*(abs(vx)^2 + abs(vy)^2 + abs(vz)^2)^(1/2)*(qw^2 - qx^2 - qy^2 + qz^2)) + vy*(2*dy*qy*(2*qw*qx + 2*qy*qz)*(abs(vx)^2 + abs(vy)^2 + abs(vz)^2)^(1/2) - 2*dx*qx*(2*qw*qy - 2*qx*qz)*(abs(vx)^2 + abs(vy)^2 + abs(vz)^2)^(1/2) - 2*dx*qw*(2*qw*qz + 2*qx*qy)*(abs(vx)^2 + abs(vy)^2 + abs(vz)^2)^(1/2) + 2*dz*qy*(2*qw*qx - 2*qy*qz)*(abs(vx)^2 + abs(vy)^2 + abs(vz)^2)^(1/2) + 2*dy*qz*(abs(vx)^2 + abs(vy)^2 + abs(vz)^2)^(1/2)*(qw^2 - qx^2 + qy^2 - qz^2) + 2*dz*qz*(abs(vx)^2 + abs(vy)^2 + abs(vz)^2)^(1/2)*(qw^2 - qx^2 - qy^2 + qz^2)) + vz*(4*dx*qw*(2*qw*qy - 2*qx*qz)*(abs(vx)^2 + abs(vy)^2 + abs(vz)^2)^(1/2) + 4*dy*qz*(2*qw*qx + 2*qy*qz)*(abs(vx)^2 + abs(vy)^2 + abs(vz)^2)^(1/2) - 4*dz*qy*(abs(vx)^2 + abs(vy)^2 + abs(vz)^2)^(1/2)*(qw^2 - qx^2 - qy^2 + qz^2))))/(abs(qw)^2 + abs(qx)^2 + abs(qy)^2 + abs(qz)^2)^(3/2) - (qw*qz*(vx*(2*dx*qz*(2*qw*qy - 2*qx*qz)*(abs(vx)^2 + abs(vy)^2 + abs(vz)^2)^(1/2) - 2*dy*qw*(2*qw*qx + 2*qy*qz)*(abs(vx)^2 + abs(vy)^2 + abs(vz)^2)^(1/2) - 2*dy*qy*(2*qw*qz - 2*qx*qy)*(abs(vx)^2 + abs(vy)^2 + abs(vz)^2)^(1/2) + 2*dz*qz*(2*qw*qy + 2*qx*qz)*(abs(vx)^2 + abs(vy)^2 + abs(vz)^2)^(1/2) + 2*dx*qx*(abs(vx)^2 + abs(vy)^2 + abs(vz)^2)^(1/2)*(qw^2 + qx^2 - qy^2 - qz^2) + 2*dz*qx*(abs(vx)^2 + abs(vy)^2 + abs(vz)^2)^(1/2)*(qw^2 - qx^2 - qy^2 + qz^2)) - vy*(2*dx*qw*(2*qw*qy - 2*qx*qz)*(abs(vx)^2 + abs(vy)^2 + abs(vz)^2)^(1/2) - 2*dx*qx*(2*qw*qz + 2*qx*qy)*(abs(vx)^2 + abs(vy)^2 + abs(vz)^2)^(1/2) + 2*dy*qz*(2*qw*qx + 2*qy*qz)*(abs(vx)^2 + abs(vy)^2 + abs(vz)^2)^(1/2) + 2*dz*qz*(2*qw*qx - 2*qy*qz)*(abs(vx)^2 + abs(vy)^2 + abs(vz)^2)^(1/2) - 2*dy*qy*(abs(vx)^2 + abs(vy)^2 + abs(vz)^2)^(1/2)*(qw^2 - qx^2 + qy^2 - qz^2) - 2*dz*qy*(abs(vx)^2 + abs(vy)^2 + abs(vz)^2)^(1/2)*(qw^2 - qx^2 - qy^2 + qz^2)) + vz*(4*dy*qy*(2*qw*qx + 2*qy*qz)*(abs(vx)^2 + abs(vy)^2 + abs(vz)^2)^(1/2) - 4*dx*qx*(2*qw*qy - 2*qx*qz)*(abs(vx)^2 + abs(vy)^2 + abs(vz)^2)^(1/2) + 4*dz*qz*(abs(vx)^2 + abs(vy)^2 + abs(vz)^2)^(1/2)*(qw^2 - qx^2 - qy^2 + qz^2))))/(abs(qw)^2 + abs(qx)^2 + abs(qy)^2 + abs(qz)^2)^(3/2), ((qx^2/(abs(qw)^2 + abs(qx)^2 + abs(qy)^2 + abs(qz)^2) - 1)*(vy*(2*dx*qy*(2*qw*qy - 2*qx*qz)*(abs(vx)^2 + abs(vy)^2 + abs(vz)^2)^(1/2) + 2*dy*qx*(2*qw*qx + 2*qy*qz)*(abs(vx)^2 + abs(vy)^2 + abs(vz)^2)^(1/2) - 2*dx*qz*(2*qw*qz + 2*qx*qy)*(abs(vx)^2 + abs(vy)^2 + abs(vz)^2)^(1/2) - 2*dz*qx*(2*qw*qx - 2*qy*qz)*(abs(vx)^2 + abs(vy)^2 + abs(vz)^2)^(1/2) - 2*dy*qw*(abs(vx)^2 + abs(vy)^2 + abs(vz)^2)^(1/2)*(qw^2 - qx^2 + qy^2 - qz^2) + 2*dz*qw*(abs(vx)^2 + abs(vy)^2 + abs(vz)^2)^(1/2)*(qw^2 - qx^2 - qy^2 + qz^2)) + vx*(2*dx*qx*(2*qw*qy - 2*qx*qz)*(abs(vx)^2 + abs(vy)^2 + abs(vz)^2)^(1/2) + 2*dy*qw*(2*qw*qz - 2*qx*qy)*(abs(vx)^2 + abs(vy)^2 + abs(vz)^2)^(1/2) - 2*dy*qy*(2*qw*qx + 2*qy*qz)*(abs(vx)^2 + abs(vy)^2 + abs(vz)^2)^(1/2) + 2*dz*qx*(2*qw*qy + 2*qx*qz)*(abs(vx)^2 + abs(vy)^2 + abs(vz)^2)^(1/2) - 2*dx*qz*(abs(vx)^2 + abs(vy)^2 + abs(vz)^2)^(1/2)*(qw^2 + qx^2 - qy^2 - qz^2) - 2*dz*qz*(abs(vx)^2 + abs(vy)^2 + abs(vz)^2)^(1/2)*(qw^2 - qx^2 - qy^2 + qz^2)) + vz*(4*dx*qz*(2*qw*qy - 2*qx*qz)*(abs(vx)^2 + abs(vy)^2 + abs(vz)^2)^(1/2) - 4*dy*qw*(2*qw*qx + 2*qy*qz)*(abs(vx)^2 + abs(vy)^2 + abs(vz)^2)^(1/2) + 4*dz*qx*(abs(vx)^2 + abs(vy)^2 + abs(vz)^2)^(1/2)*(qw^2 - qx^2 - qy^2 + qz^2))))/(abs(qw)^2 + abs(qx)^2 + abs(qy)^2 + abs(qz)^2)^(1/2) + (qw*qx*(vx*(2*dx*qw*(2*qw*qy - 2*qx*qz)*(abs(vx)^2 + abs(vy)^2 + abs(vz)^2)^(1/2) + 2*dy*qx*(2*qw*qz - 2*qx*qy)*(abs(vx)^2 + abs(vy)^2 + abs(vz)^2)^(1/2) - 2*dz*qw*(2*qw*qy + 2*qx*qz)*(abs(vx)^2 + abs(vy)^2 + abs(vz)^2)^(1/2) + 2*dy*qz*(2*qw*qx + 2*qy*qz)*(abs(vx)^2 + abs(vy)^2 + abs(vz)^2)^(1/2) + 2*dx*qy*(abs(vx)^2 + abs(vy)^2 + abs(vz)^2)^(1/2)*(qw^2 + qx^2 - qy^2 - qz^2) - 2*dz*qy*(abs(vx)^2 + abs(vy)^2 + abs(vz)^2)^(1/2)*(qw^2 - qx^2 - qy^2 + qz^2)) + vy*(2*dx*qy*(2*qw*qz + 2*qx*qy)*(abs(vx)^2 + abs(vy)^2 + abs(vz)^2)^(1/2) - 2*dy*qw*(2*qw*qx + 2*qy*qz)*(abs(vx)^2 + abs(vy)^2 + abs(vz)^2)^(1/2) + 2*dz*qw*(2*qw*qx - 2*qy*qz)*(abs(vx)^2 + abs(vy)^2 + abs(vz)^2)^(1/2) + 2*dx*qz*(2*qw*qy - 2*qx*qz)*(abs(vx)^2 + abs(vy)^2 + abs(vz)^2)^(1/2) - 2*dy*qx*(abs(vx)^2 + abs(vy)^2 + abs(vz)^2)^(1/2)*(qw^2 - qx^2 + qy^2 - qz^2) + 2*dz*qx*(abs(vx)^2 + abs(vy)^2 + abs(vz)^2)^(1/2)*(qw^2 - qx^2 - qy^2 + qz^2)) - vz*(4*dx*qy*(2*qw*qy - 2*qx*qz)*(abs(vx)^2 + abs(vy)^2 + abs(vz)^2)^(1/2) + 4*dy*qx*(2*qw*qx + 2*qy*qz)*(abs(vx)^2 + abs(vy)^2 + abs(vz)^2)^(1/2) + 4*dz*qw*(abs(vx)^2 + abs(vy)^2 + abs(vz)^2)^(1/2)*(qw^2 - qx^2 - qy^2 + qz^2))))/(abs(qw)^2 + abs(qx)^2 + abs(qy)^2 + abs(qz)^2)^(3/2) - (qx*qy*(vx*(2*dx*qy*(2*qw*qy - 2*qx*qz)*(abs(vx)^2 + abs(vy)^2 + abs(vz)^2)^(1/2) + 2*dy*qx*(2*qw*qx + 2*qy*qz)*(abs(vx)^2 + abs(vy)^2 + abs(vz)^2)^(1/2) - 2*dy*qz*(2*qw*qz - 2*qx*qy)*(abs(vx)^2 + abs(vy)^2 + abs(vz)^2)^(1/2) - 2*dz*qy*(2*qw*qy + 2*qx*qz)*(abs(vx)^2 + abs(vy)^2 + abs(vz)^2)^(1/2) - 2*dx*qw*(abs(vx)^2 + abs(vy)^2 + abs(vz)^2)^(1/2)*(qw^2 + qx^2 - qy^2 - qz^2) + 2*dz*qw*(abs(vx)^2 + abs(vy)^2 + abs(vz)^2)^(1/2)*(qw^2 - qx^2 - qy^2 + qz^2)) + vy*(2*dy*qy*(2*qw*qx + 2*qy*qz)*(abs(vx)^2 + abs(vy)^2 + abs(vz)^2)^(1/2) - 2*dx*qx*(2*qw*qy - 2*qx*qz)*(abs(vx)^2 + abs(vy)^2 + abs(vz)^2)^(1/2) - 2*dx*qw*(2*qw*qz + 2*qx*qy)*(abs(vx)^2 + abs(vy)^2 + abs(vz)^2)^(1/2) + 2*dz*qy*(2*qw*qx - 2*qy*qz)*(abs(vx)^2 + abs(vy)^2 + abs(vz)^2)^(1/2) + 2*dy*qz*(abs(vx)^2 + abs(vy)^2 + abs(vz)^2)^(1/2)*(qw^2 - qx^2 + qy^2 - qz^2) + 2*dz*qz*(abs(vx)^2 + abs(vy)^2 + abs(vz)^2)^(1/2)*(qw^2 - qx^2 - qy^2 + qz^2)) + vz*(4*dx*qw*(2*qw*qy - 2*qx*qz)*(abs(vx)^2 + abs(vy)^2 + abs(vz)^2)^(1/2) + 4*dy*qz*(2*qw*qx + 2*qy*qz)*(abs(vx)^2 + abs(vy)^2 + abs(vz)^2)^(1/2) - 4*dz*qy*(abs(vx)^2 + abs(vy)^2 + abs(vz)^2)^(1/2)*(qw^2 - qx^2 - qy^2 + qz^2))))/(abs(qw)^2 + abs(qx)^2 + abs(qy)^2 + abs(qz)^2)^(3/2) - (qx*qz*(vx*(2*dx*qz*(2*qw*qy - 2*qx*qz)*(abs(vx)^2 + abs(vy)^2 + abs(vz)^2)^(1/2) - 2*dy*qw*(2*qw*qx + 2*qy*qz)*(abs(vx)^2 + abs(vy)^2 + abs(vz)^2)^(1/2) - 2*dy*qy*(2*qw*qz - 2*qx*qy)*(abs(vx)^2 + abs(vy)^2 + abs(vz)^2)^(1/2) + 2*dz*qz*(2*qw*qy + 2*qx*qz)*(abs(vx)^2 + abs(vy)^2 + abs(vz)^2)^(1/2) + 2*dx*qx*(abs(vx)^2 + abs(vy)^2 + abs(vz)^2)^(1/2)*(qw^2 + qx^2 - qy^2 - qz^2) + 2*dz*qx*(abs(vx)^2 + abs(vy)^2 + abs(vz)^2)^(1/2)*(qw^2 - qx^2 - qy^2 + qz^2)) - vy*(2*dx*qw*(2*qw*qy - 2*qx*qz)*(abs(vx)^2 + abs(vy)^2 + abs(vz)^2)^(1/2) - 2*dx*qx*(2*qw*qz + 2*qx*qy)*(abs(vx)^2 + abs(vy)^2 + abs(vz)^2)^(1/2) + 2*dy*qz*(2*qw*qx + 2*qy*qz)*(abs(vx)^2 + abs(vy)^2 + abs(vz)^2)^(1/2) + 2*dz*qz*(2*qw*qx - 2*qy*qz)*(abs(vx)^2 + abs(vy)^2 + abs(vz)^2)^(1/2) - 2*dy*qy*(abs(vx)^2 + abs(vy)^2 + abs(vz)^2)^(1/2)*(qw^2 - qx^2 + qy^2 - qz^2) - 2*dz*qy*(abs(vx)^2 + abs(vy)^2 + abs(vz)^2)^(1/2)*(qw^2 - qx^2 - qy^2 + qz^2)) + vz*(4*dy*qy*(2*qw*qx + 2*qy*qz)*(abs(vx)^2 + abs(vy)^2 + abs(vz)^2)^(1/2) - 4*dx*qx*(2*qw*qy - 2*qx*qz)*(abs(vx)^2 + abs(vy)^2 + abs(vz)^2)^(1/2) + 4*dz*qz*(abs(vx)^2 + abs(vy)^2 + abs(vz)^2)^(1/2)*(qw^2 - qx^2 - qy^2 + qz^2))))/(abs(qw)^2 + abs(qx)^2 + abs(qy)^2 + abs(qz)^2)^(3/2), (qw*qy*(vx*(2*dx*qw*(2*qw*qy - 2*qx*qz)*(abs(vx)^2 + abs(vy)^2 + abs(vz)^2)^(1/2) + 2*dy*qx*(2*qw*qz - 2*qx*qy)*(abs(vx)^2 + abs(vy)^2 + abs(vz)^2)^(1/2) - 2*dz*qw*(2*qw*qy + 2*qx*qz)*(abs(vx)^2 + abs(vy)^2 + abs(vz)^2)^(1/2) + 2*dy*qz*(2*qw*qx + 2*qy*qz)*(abs(vx)^2 + abs(vy)^2 + abs(vz)^2)^(1/2) + 2*dx*qy*(abs(vx)^2 + abs(vy)^2 + abs(vz)^2)^(1/2)*(qw^2 + qx^2 - qy^2 - qz^2) - 2*dz*qy*(abs(vx)^2 + abs(vy)^2 + abs(vz)^2)^(1/2)*(qw^2 - qx^2 - qy^2 + qz^2)) + vy*(2*dx*qy*(2*qw*qz + 2*qx*qy)*(abs(vx)^2 + abs(vy)^2 + abs(vz)^2)^(1/2) - 2*dy*qw*(2*qw*qx + 2*qy*qz)*(abs(vx)^2 + abs(vy)^2 + abs(vz)^2)^(1/2) + 2*dz*qw*(2*qw*qx - 2*qy*qz)*(abs(vx)^2 + abs(vy)^2 + abs(vz)^2)^(1/2) + 2*dx*qz*(2*qw*qy - 2*qx*qz)*(abs(vx)^2 + abs(vy)^2 + abs(vz)^2)^(1/2) - 2*dy*qx*(abs(vx)^2 + abs(vy)^2 + abs(vz)^2)^(1/2)*(qw^2 - qx^2 + qy^2 - qz^2) + 2*dz*qx*(abs(vx)^2 + abs(vy)^2 + abs(vz)^2)^(1/2)*(qw^2 - qx^2 - qy^2 + qz^2)) - vz*(4*dx*qy*(2*qw*qy - 2*qx*qz)*(abs(vx)^2 + abs(vy)^2 + abs(vz)^2)^(1/2) + 4*dy*qx*(2*qw*qx + 2*qy*qz)*(abs(vx)^2 + abs(vy)^2 + abs(vz)^2)^(1/2) + 4*dz*qw*(abs(vx)^2 + abs(vy)^2 + abs(vz)^2)^(1/2)*(qw^2 - qx^2 - qy^2 + qz^2))))/(abs(qw)^2 + abs(qx)^2 + abs(qy)^2 + abs(qz)^2)^(3/2) - ((qy^2/(abs(qw)^2 + abs(qx)^2 + abs(qy)^2 + abs(qz)^2) - 1)*(vx*(2*dx*qy*(2*qw*qy - 2*qx*qz)*(abs(vx)^2 + abs(vy)^2 + abs(vz)^2)^(1/2) + 2*dy*qx*(2*qw*qx + 2*qy*qz)*(abs(vx)^2 + abs(vy)^2 + abs(vz)^2)^(1/2) - 2*dy*qz*(2*qw*qz - 2*qx*qy)*(abs(vx)^2 + abs(vy)^2 + abs(vz)^2)^(1/2) - 2*dz*qy*(2*qw*qy + 2*qx*qz)*(abs(vx)^2 + abs(vy)^2 + abs(vz)^2)^(1/2) - 2*dx*qw*(abs(vx)^2 + abs(vy)^2 + abs(vz)^2)^(1/2)*(qw^2 + qx^2 - qy^2 - qz^2) + 2*dz*qw*(abs(vx)^2 + abs(vy)^2 + abs(vz)^2)^(1/2)*(qw^2 - qx^2 - qy^2 + qz^2)) + vy*(2*dy*qy*(2*qw*qx + 2*qy*qz)*(abs(vx)^2 + abs(vy)^2 + abs(vz)^2)^(1/2) - 2*dx*qx*(2*qw*qy - 2*qx*qz)*(abs(vx)^2 + abs(vy)^2 + abs(vz)^2)^(1/2) - 2*dx*qw*(2*qw*qz + 2*qx*qy)*(abs(vx)^2 + abs(vy)^2 + abs(vz)^2)^(1/2) + 2*dz*qy*(2*qw*qx - 2*qy*qz)*(abs(vx)^2 + abs(vy)^2 + abs(vz)^2)^(1/2) + 2*dy*qz*(abs(vx)^2 + abs(vy)^2 + abs(vz)^2)^(1/2)*(qw^2 - qx^2 + qy^2 - qz^2) + 2*dz*qz*(abs(vx)^2 + abs(vy)^2 + abs(vz)^2)^(1/2)*(qw^2 - qx^2 - qy^2 + qz^2)) + vz*(4*dx*qw*(2*qw*qy - 2*qx*qz)*(abs(vx)^2 + abs(vy)^2 + abs(vz)^2)^(1/2) + 4*dy*qz*(2*qw*qx + 2*qy*qz)*(abs(vx)^2 + abs(vy)^2 + abs(vz)^2)^(1/2) - 4*dz*qy*(abs(vx)^2 + abs(vy)^2 + abs(vz)^2)^(1/2)*(qw^2 - qx^2 - qy^2 + qz^2))))/(abs(qw)^2 + abs(qx)^2 + abs(qy)^2 + abs(qz)^2)^(1/2) + (qx*qy*(vy*(2*dx*qy*(2*qw*qy - 2*qx*qz)*(abs(vx)^2 + abs(vy)^2 + abs(vz)^2)^(1/2) + 2*dy*qx*(2*qw*qx + 2*qy*qz)*(abs(vx)^2 + abs(vy)^2 + abs(vz)^2)^(1/2) - 2*dx*qz*(2*qw*qz + 2*qx*qy)*(abs(vx)^2 + abs(vy)^2 + abs(vz)^2)^(1/2) - 2*dz*qx*(2*qw*qx - 2*qy*qz)*(abs(vx)^2 + abs(vy)^2 + abs(vz)^2)^(1/2) - 2*dy*qw*(abs(vx)^2 + abs(vy)^2 + abs(vz)^2)^(1/2)*(qw^2 - qx^2 + qy^2 - qz^2) + 2*dz*qw*(abs(vx)^2 + abs(vy)^2 + abs(vz)^2)^(1/2)*(qw^2 - qx^2 - qy^2 + qz^2)) + vx*(2*dx*qx*(2*qw*qy - 2*qx*qz)*(abs(vx)^2 + abs(vy)^2 + abs(vz)^2)^(1/2) + 2*dy*qw*(2*qw*qz - 2*qx*qy)*(abs(vx)^2 + abs(vy)^2 + abs(vz)^2)^(1/2) - 2*dy*qy*(2*qw*qx + 2*qy*qz)*(abs(vx)^2 + abs(vy)^2 + abs(vz)^2)^(1/2) + 2*dz*qx*(2*qw*qy + 2*qx*qz)*(abs(vx)^2 + abs(vy)^2 + abs(vz)^2)^(1/2) - 2*dx*qz*(abs(vx)^2 + abs(vy)^2 + abs(vz)^2)^(1/2)*(qw^2 + qx^2 - qy^2 - qz^2) - 2*dz*qz*(abs(vx)^2 + abs(vy)^2 + abs(vz)^2)^(1/2)*(qw^2 - qx^2 - qy^2 + qz^2)) + vz*(4*dx*qz*(2*qw*qy - 2*qx*qz)*(abs(vx)^2 + abs(vy)^2 + abs(vz)^2)^(1/2) - 4*dy*qw*(2*qw*qx + 2*qy*qz)*(abs(vx)^2 + abs(vy)^2 + abs(vz)^2)^(1/2) + 4*dz*qx*(abs(vx)^2 + abs(vy)^2 + abs(vz)^2)^(1/2)*(qw^2 - qx^2 - qy^2 + qz^2))))/(abs(qw)^2 + abs(qx)^2 + abs(qy)^2 + abs(qz)^2)^(3/2) - (qy*qz*(vx*(2*dx*qz*(2*qw*qy - 2*qx*qz)*(abs(vx)^2 + abs(vy)^2 + abs(vz)^2)^(1/2) - 2*dy*qw*(2*qw*qx + 2*qy*qz)*(abs(vx)^2 + abs(vy)^2 + abs(vz)^2)^(1/2) - 2*dy*qy*(2*qw*qz - 2*qx*qy)*(abs(vx)^2 + abs(vy)^2 + abs(vz)^2)^(1/2) + 2*dz*qz*(2*qw*qy + 2*qx*qz)*(abs(vx)^2 + abs(vy)^2 + abs(vz)^2)^(1/2) + 2*dx*qx*(abs(vx)^2 + abs(vy)^2 + abs(vz)^2)^(1/2)*(qw^2 + qx^2 - qy^2 - qz^2) + 2*dz*qx*(abs(vx)^2 + abs(vy)^2 + abs(vz)^2)^(1/2)*(qw^2 - qx^2 - qy^2 + qz^2)) - vy*(2*dx*qw*(2*qw*qy - 2*qx*qz)*(abs(vx)^2 + abs(vy)^2 + abs(vz)^2)^(1/2) - 2*dx*qx*(2*qw*qz + 2*qx*qy)*(abs(vx)^2 + abs(vy)^2 + abs(vz)^2)^(1/2) + 2*dy*qz*(2*qw*qx + 2*qy*qz)*(abs(vx)^2 + abs(vy)^2 + abs(vz)^2)^(1/2) + 2*dz*qz*(2*qw*qx - 2*qy*qz)*(abs(vx)^2 + abs(vy)^2 + abs(vz)^2)^(1/2) - 2*dy*qy*(abs(vx)^2 + abs(vy)^2 + abs(vz)^2)^(1/2)*(qw^2 - qx^2 + qy^2 - qz^2) - 2*dz*qy*(abs(vx)^2 + abs(vy)^2 + abs(vz)^2)^(1/2)*(qw^2 - qx^2 - qy^2 + qz^2)) + vz*(4*dy*qy*(2*qw*qx + 2*qy*qz)*(abs(vx)^2 + abs(vy)^2 + abs(vz)^2)^(1/2) - 4*dx*qx*(2*qw*qy - 2*qx*qz)*(abs(vx)^2 + abs(vy)^2 + abs(vz)^2)^(1/2) + 4*dz*qz*(abs(vx)^2 + abs(vy)^2 + abs(vz)^2)^(1/2)*(qw^2 - qx^2 - qy^2 + qz^2))))/(abs(qw)^2 + abs(qx)^2 + abs(qy)^2 + abs(qz)^2)^(3/2), (qw*qz*(vx*(2*dx*qw*(2*qw*qy - 2*qx*qz)*(abs(vx)^2 + abs(vy)^2 + abs(vz)^2)^(1/2) + 2*dy*qx*(2*qw*qz - 2*qx*qy)*(abs(vx)^2 + abs(vy)^2 + abs(vz)^2)^(1/2) - 2*dz*qw*(2*qw*qy + 2*qx*qz)*(abs(vx)^2 + abs(vy)^2 + abs(vz)^2)^(1/2) + 2*dy*qz*(2*qw*qx + 2*qy*qz)*(abs(vx)^2 + abs(vy)^2 + abs(vz)^2)^(1/2) + 2*dx*qy*(abs(vx)^2 + abs(vy)^2 + abs(vz)^2)^(1/2)*(qw^2 + qx^2 - qy^2 - qz^2) - 2*dz*qy*(abs(vx)^2 + abs(vy)^2 + abs(vz)^2)^(1/2)*(qw^2 - qx^2 - qy^2 + qz^2)) + vy*(2*dx*qy*(2*qw*qz + 2*qx*qy)*(abs(vx)^2 + abs(vy)^2 + abs(vz)^2)^(1/2) - 2*dy*qw*(2*qw*qx + 2*qy*qz)*(abs(vx)^2 + abs(vy)^2 + abs(vz)^2)^(1/2) + 2*dz*qw*(2*qw*qx - 2*qy*qz)*(abs(vx)^2 + abs(vy)^2 + abs(vz)^2)^(1/2) + 2*dx*qz*(2*qw*qy - 2*qx*qz)*(abs(vx)^2 + abs(vy)^2 + abs(vz)^2)^(1/2) - 2*dy*qx*(abs(vx)^2 + abs(vy)^2 + abs(vz)^2)^(1/2)*(qw^2 - qx^2 + qy^2 - qz^2) + 2*dz*qx*(abs(vx)^2 + abs(vy)^2 + abs(vz)^2)^(1/2)*(qw^2 - qx^2 - qy^2 + qz^2)) - vz*(4*dx*qy*(2*qw*qy - 2*qx*qz)*(abs(vx)^2 + abs(vy)^2 + abs(vz)^2)^(1/2) + 4*dy*qx*(2*qw*qx + 2*qy*qz)*(abs(vx)^2 + abs(vy)^2 + abs(vz)^2)^(1/2) + 4*dz*qw*(abs(vx)^2 + abs(vy)^2 + abs(vz)^2)^(1/2)*(qw^2 - qx^2 - qy^2 + qz^2))))/(abs(qw)^2 + abs(qx)^2 + abs(qy)^2 + abs(qz)^2)^(3/2) - ((qz^2/(abs(qw)^2 + abs(qx)^2 + abs(qy)^2 + abs(qz)^2) - 1)*(vx*(2*dx*qz*(2*qw*qy - 2*qx*qz)*(abs(vx)^2 + abs(vy)^2 + abs(vz)^2)^(1/2) - 2*dy*qw*(2*qw*qx + 2*qy*qz)*(abs(vx)^2 + abs(vy)^2 + abs(vz)^2)^(1/2) - 2*dy*qy*(2*qw*qz - 2*qx*qy)*(abs(vx)^2 + abs(vy)^2 + abs(vz)^2)^(1/2) + 2*dz*qz*(2*qw*qy + 2*qx*qz)*(abs(vx)^2 + abs(vy)^2 + abs(vz)^2)^(1/2) + 2*dx*qx*(abs(vx)^2 + abs(vy)^2 + abs(vz)^2)^(1/2)*(qw^2 + qx^2 - qy^2 - qz^2) + 2*dz*qx*(abs(vx)^2 + abs(vy)^2 + abs(vz)^2)^(1/2)*(qw^2 - qx^2 - qy^2 + qz^2)) - vy*(2*dx*qw*(2*qw*qy - 2*qx*qz)*(abs(vx)^2 + abs(vy)^2 + abs(vz)^2)^(1/2) - 2*dx*qx*(2*qw*qz + 2*qx*qy)*(abs(vx)^2 + abs(vy)^2 + abs(vz)^2)^(1/2) + 2*dy*qz*(2*qw*qx + 2*qy*qz)*(abs(vx)^2 + abs(vy)^2 + abs(vz)^2)^(1/2) + 2*dz*qz*(2*qw*qx - 2*qy*qz)*(abs(vx)^2 + abs(vy)^2 + abs(vz)^2)^(1/2) - 2*dy*qy*(abs(vx)^2 + abs(vy)^2 + abs(vz)^2)^(1/2)*(qw^2 - qx^2 + qy^2 - qz^2) - 2*dz*qy*(abs(vx)^2 + abs(vy)^2 + abs(vz)^2)^(1/2)*(qw^2 - qx^2 - qy^2 + qz^2)) + vz*(4*dy*qy*(2*qw*qx + 2*qy*qz)*(abs(vx)^2 + abs(vy)^2 + abs(vz)^2)^(1/2) - 4*dx*qx*(2*qw*qy - 2*qx*qz)*(abs(vx)^2 + abs(vy)^2 + abs(vz)^2)^(1/2) + 4*dz*qz*(abs(vx)^2 + abs(vy)^2 + abs(vz)^2)^(1/2)*(qw^2 - qx^2 - qy^2 + qz^2))))/(abs(qw)^2 + abs(qx)^2 + abs(qy)^2 + abs(qz)^2)^(1/2) + (qx*qz*(vy*(2*dx*qy*(2*qw*qy - 2*qx*qz)*(abs(vx)^2 + abs(vy)^2 + abs(vz)^2)^(1/2) + 2*dy*qx*(2*qw*qx + 2*qy*qz)*(abs(vx)^2 + abs(vy)^2 + abs(vz)^2)^(1/2) - 2*dx*qz*(2*qw*qz + 2*qx*qy)*(abs(vx)^2 + abs(vy)^2 + abs(vz)^2)^(1/2) - 2*dz*qx*(2*qw*qx - 2*qy*qz)*(abs(vx)^2 + abs(vy)^2 + abs(vz)^2)^(1/2) - 2*dy*qw*(abs(vx)^2 + abs(vy)^2 + abs(vz)^2)^(1/2)*(qw^2 - qx^2 + qy^2 - qz^2) + 2*dz*qw*(abs(vx)^2 + abs(vy)^2 + abs(vz)^2)^(1/2)*(qw^2 - qx^2 - qy^2 + qz^2)) + vx*(2*dx*qx*(2*qw*qy - 2*qx*qz)*(abs(vx)^2 + abs(vy)^2 + abs(vz)^2)^(1/2) + 2*dy*qw*(2*qw*qz - 2*qx*qy)*(abs(vx)^2 + abs(vy)^2 + abs(vz)^2)^(1/2) - 2*dy*qy*(2*qw*qx + 2*qy*qz)*(abs(vx)^2 + abs(vy)^2 + abs(vz)^2)^(1/2) + 2*dz*qx*(2*qw*qy + 2*qx*qz)*(abs(vx)^2 + abs(vy)^2 + abs(vz)^2)^(1/2) - 2*dx*qz*(abs(vx)^2 + abs(vy)^2 + abs(vz)^2)^(1/2)*(qw^2 + qx^2 - qy^2 - qz^2) - 2*dz*qz*(abs(vx)^2 + abs(vy)^2 + abs(vz)^2)^(1/2)*(qw^2 - qx^2 - qy^2 + qz^2)) + vz*(4*dx*qz*(2*qw*qy - 2*qx*qz)*(abs(vx)^2 + abs(vy)^2 + abs(vz)^2)^(1/2) - 4*dy*qw*(2*qw*qx + 2*qy*qz)*(abs(vx)^2 + abs(vy)^2 + abs(vz)^2)^(1/2) + 4*dz*qx*(abs(vx)^2 + abs(vy)^2 + abs(vz)^2)^(1/2)*(qw^2 - qx^2 - qy^2 + qz^2))))/(abs(qw)^2 + abs(qx)^2 + abs(qy)^2 + abs(qz)^2)^(3/2) - (qy*qz*(vx*(2*dx*qy*(2*qw*qy - 2*qx*qz)*(abs(vx)^2 + abs(vy)^2 + abs(vz)^2)^(1/2) + 2*dy*qx*(2*qw*qx + 2*qy*qz)*(abs(vx)^2 + abs(vy)^2 + abs(vz)^2)^(1/2) - 2*dy*qz*(2*qw*qz - 2*qx*qy)*(abs(vx)^2 + abs(vy)^2 + abs(vz)^2)^(1/2) - 2*dz*qy*(2*qw*qy + 2*qx*qz)*(abs(vx)^2 + abs(vy)^2 + abs(vz)^2)^(1/2) - 2*dx*qw*(abs(vx)^2 + abs(vy)^2 + abs(vz)^2)^(1/2)*(qw^2 + qx^2 - qy^2 - qz^2) + 2*dz*qw*(abs(vx)^2 + abs(vy)^2 + abs(vz)^2)^(1/2)*(qw^2 - qx^2 - qy^2 + qz^2)) + vy*(2*dy*qy*(2*qw*qx + 2*qy*qz)*(abs(vx)^2 + abs(vy)^2 + abs(vz)^2)^(1/2) - 2*dx*qx*(2*qw*qy - 2*qx*qz)*(abs(vx)^2 + abs(vy)^2 + abs(vz)^2)^(1/2) - 2*dx*qw*(2*qw*qz + 2*qx*qy)*(abs(vx)^2 + abs(vy)^2 + abs(vz)^2)^(1/2) + 2*dz*qy*(2*qw*qx - 2*qy*qz)*(abs(vx)^2 + abs(vy)^2 + abs(vz)^2)^(1/2) + 2*dy*qz*(abs(vx)^2 + abs(vy)^2 + abs(vz)^2)^(1/2)*(qw^2 - qx^2 + qy^2 - qz^2) + 2*dz*qz*(abs(vx)^2 + abs(vy)^2 + abs(vz)^2)^(1/2)*(qw^2 - qx^2 - qy^2 + qz^2)) + vz*(4*dx*qw*(2*qw*qy - 2*qx*qz)*(abs(vx)^2 + abs(vy)^2 + abs(vz)^2)^(1/2) + 4*dy*qz*(2*qw*qx + 2*qy*qz)*(abs(vx)^2 + abs(vy)^2 + abs(vz)^2)^(1/2) - 4*dz*qy*(abs(vx)^2 + abs(vy)^2 + abs(vz)^2)^(1/2)*(qw^2 - qx^2 - qy^2 + qz^2))))/(abs(qw)^2 + abs(qx)^2 + abs(qy)^2 + abs(qz)^2)^(3/2)];
%  
ddv_dq=-(ddc_dq)/m;

A = [zeros(3),   zeros(3,4), ddp_dv;...
     zeros(4,3), ddq_dq,     zeros(4,3);...
     zeros(3) ,  ddv_dq,     zeros(3)];
B = [zeros(3), zeros(3,1);...
       ddq_dw, zeros(4,1);...
       zeros(3),    ddv_dc];
   
   
Q=P.Q; R=P.R;

K0 = lqr(A,B,Q,R);
% uref = [0;0;0;0];          % Hao
y= uref+(-K0*(x_c-xref));  %desired omegas and fc



for i=1:3
    if y(i)>1.5
        y(i)=1.5;
    elseif y(i)<-1.5
        y(i)=-1.5;
    end
end
